simulink model "lss"  (R2022b)
settings: Solver=FixedStepAuto  StartTime=0.0  StopTime=Inf  FixedStep=0.001  RelTol=1e-3  EnableMultiTasking=on
InitFcn:
  | clear mex
model workspace (MAT data in the model file):
  worldsim_instance : object (value not decoded)
values from neighbouring files (symbols this model uses):
  ADAS_Control_Mode = 1    [LSS_parameters.m]    (also in lss_ini_param.sldd = 1.0)
  butter_a = 1.0 -1.9911142922016536 0.99115359586893548    [lss_ini_param.sldd]
  butter_a_lka_out = 1.0 -1.5610180758007179 0.641351538057563    [lss_ini_param.sldd]
  butter_b = 9.825916820482009E-6 1.9651833640964018E-5 9.825916820482009E-6    [lss_ini_param.sldd]
  butter_b_lka_out = 0.020083365564211246 0.040166731128422492 0.020083365564211246    [lss_ini_param.sldd]
  index_variant_approaching_speed = 3.0    [lss_ini_param.sldd]
  initCond = vi_worldsim_load_scenario(worldsim_process,scenario_path,'lss_online')    [launcher.m]
  LDW_Activity_Flag = 1    [LSS_parameters.m]    (also in lss_ini_param.sldd = 1.0)
  LDW_Freq_Hz = Sensor_Freq_worldsim    [LSS_parameters.m]    (also in lss_ini_param.sldd = 50.0)
  LDW_LaneGap_dydt_Warning = 50    [LSS_parameters.m]    (also in lss_ini_param.sldd = 50.0)
  LDW_LaneGap_Warning = [0.5 0.25]    [LSS_parameters.m]    (also in lss_ini_param.sldd = 0.5 0.25)
  LDW_Min_Speed = 60    [LSS_parameters.m]    (also in lss_ini_param.sldd = 60.0)
  LDW_Steer_Vibration_Amplitude = 5    [LSS_parameters.m]    (also in lss_ini_param.sldd = 5.0)
  LDW_Steer_Vibration_Freq = 25    [LSS_parameters.m]    (also in lss_ini_param.sldd = 25.0)
  LKA_Activity_Flag = 1    [LSS_parameters.m]    (also in lss_ini_param.sldd = 1.0)
  LKA_D = [0.2 0.3]    [LSS_parameters.m]    (also in lss_ini_param.sldd = 0.2 0.3)
  LKA_Dyn_Rate_Limiter_Gain = 0.1    [LSS_parameters.m]    (also in lss_ini_param.sldd)
  LKA_Dyn_Rate_Limiter_Power = 10    [LSS_parameters.m]    (also in lss_ini_param.sldd = 10.0)
  LKA_Error_dydt_Off = 1    [LSS_parameters.m]    (also in lss_ini_param.sldd = 1.0)
  LKA_Error_Max = 3    [LSS_parameters.m]    (also in lss_ini_param.sldd = 3.0)
  LKA_Error_Off = 0.5    [LSS_parameters.m]    (also in lss_ini_param.sldd)
  LKA_Freq_Hz = Sensor_Freq_worldsim    [LSS_parameters.m]    (also in lss_ini_param.sldd = 50.0)
  LKA_I = [0.025 0.05]    [LSS_parameters.m]    (also in lss_ini_param.sldd = 0.025 0.05)
  LKA_Lane_Gap_Activate = [0.25 0.125]    [LSS_parameters.m]    (also in lss_ini_param.sldd = -0.05 0.125)
  LKA_Lane_Gap_dydt_Activate = 50    [LSS_parameters.m]    (also in lss_ini_param.sldd = 50.0)
  LKA_Min_Speed = 60    [LSS_parameters.m]    (also in lss_ini_param.mat = 50; lss_ini_param.sldd = 50.0)
  LKA_On_Display_Freq = 5    [LSS_parameters.m]    (also in lss_ini_param.sldd = 5.0)
  LKA_P = [0.1 0.2]    [LSS_parameters.m]    (also in lss_ini_param.sldd = 0.1 0.2)
  LKA_Steer_Rate_Max_radps = 1    [LSS_parameters.m]    (also in lss_ini_param.sldd = 1.0)
  radar_source = 2    [LSS_parameters.m]    (also in lss_ini_param.sldd = 2.0)
  Sensor_Freq_worldsim = 50    [launcher.m]    (also in lss_ini_param.sldd = 50.0)
  simulation_crt = '../VI-CarRealTime_model/SedanCar_WorldSim_Offline_send_svm.xml'    [launcher.m]
  stop_number_collisions = 5    [launcher.m]
  stop_speed = 0.001    [launcher.m]
  stop_time = 20    [launcher.m]
  target_speed = 72    [LSS_parameters.m]    (also in launcher.m = initCond.initialVelocity * 3.6)
  variant_approaching_speed = v_lat    [launcher.m]    (also in lss_ini_param.sldd = 0.2 0.3 0.4 0.5 0.6)
  vehicle_width = 1.86    [LSS_parameters.m]    (also in lss_ini_param.sldd = 2.05)
undefined symbols (not defined in the file or in its folder): Driver_Demands, light_brake_center, light_brake_left, light_brake_right, steer_assist, vicrt_initcallback, vicrt_initmexcallback, vicrt_simulationmanager
libraries: simulink x39, simwbSfunlib x15, viworldsim_lib x5
(part 4 of 6)

== system lss/VI-CarRealTime/Output_Bus/adapter ==
  inputBus : Inport
  adaBCre : BusCreator  Inputs=1353
  adaDemux : Demux  Outputs=1353
  adaSel : BusToVector
  outputBus : Outport
  wires:
  inputBus/1 -> adaSel/1
  adaSel/1 -> adaDemux/1
  adaDemux/1 -> adaBCre/1  "aero_forces:aero_balance"
  adaDemux/2 -> adaBCre/2  "aero_forces:center_downforce"
  adaDemux/3 -> adaBCre/3  "aero_forces:center_sideforce"
  adaDemux/4 -> adaBCre/4  "aero_forces:drag_arm"
  adaDemux/5 -> adaBCre/5  "aero_forces:drag_force"
  adaDemux/6 -> adaBCre/6  "aero_forces:drag_force_front"
  adaDemux/7 -> adaBCre/7  "aero_forces:drag_force_rear"
  adaDemux/8 -> adaBCre/8  "aero_forces:drag_torque"
  adaDemux/9 -> adaBCre/9  "aero_forces:front_downforce"
  adaDemux/10 -> adaBCre/10  "aero_forces:front_sideforce"
  adaDemux/11 -> adaBCre/11  "aero_forces:height_auxiliary"
  adaDemux/12 -> adaBCre/12  "aero_forces:height_front"
  adaDemux/13 -> adaBCre/13  "aero_forces:height_rear"
  adaDemux/14 -> adaBCre/14  "aero_forces:lateral_velocity"
  adaDemux/15 -> adaBCre/15  "aero_forces:longitudinal_velocity"
  adaDemux/16 -> adaBCre/16  "aero_forces:pitch"
  adaDemux/17 -> adaBCre/17  "aero_forces:rear_downforce"
  adaDemux/18 -> adaBCre/18  "aero_forces:rear_sideforce"
  adaDemux/19 -> adaBCre/19  "aero_forces:roll"
  adaDemux/20 -> adaBCre/20  "aero_forces:roll_torque"
  adaDemux/21 -> adaBCre/21  "aero_forces:side_slip"
  adaDemux/22 -> adaBCre/22  "aero_forces:steer"
  adaDemux/23 -> adaBCre/23  "aero_forces:vertical_velocity"
  adaDemux/24 -> adaBCre/24  "aero_forces:yaw_torque"
  adaDemux/25 -> adaBCre/25  "Brake:ABS_Activity:L1"
  adaDemux/26 -> adaBCre/26  "Brake:ABS_Activity:L2"
  adaDemux/27 -> adaBCre/27  "Brake:ABS_Activity:R1"
  adaDemux/28 -> adaBCre/28  "Brake:ABS_Activity:R2"
  adaDemux/29 -> adaBCre/29  "Brake:Brake_Moment:L1"
  adaDemux/30 -> adaBCre/30  "Brake:Brake_Moment:L2"
  adaDemux/31 -> adaBCre/31  "Brake:Brake_Moment:R1"
  adaDemux/32 -> adaBCre/32  "Brake:Brake_Moment:R2"
  adaDemux/33 -> adaBCre/33  "Brake:Chamber_Pressure:L1"
  adaDemux/34 -> adaBCre/34  "Brake:Chamber_Pressure:L2"
  adaDemux/35 -> adaBCre/35  "Brake:Chamber_Pressure:R1"
  adaDemux/36 -> adaBCre/36  "Brake:Chamber_Pressure:R2"
  adaDemux/37 -> adaBCre/37  "Brake:Locked_Damper_Moment:L1"
  adaDemux/38 -> adaBCre/38  "Brake:Locked_Damper_Moment:L2"
  adaDemux/39 -> adaBCre/39  "Brake:Locked_Damper_Moment:R1"
  adaDemux/40 -> adaBCre/40  "Brake:Locked_Damper_Moment:R2"
  adaDemux/41 -> adaBCre/41  "Brake:Locked_Moment:L1"
  adaDemux/42 -> adaBCre/42  "Brake:Locked_Moment:L2"
  adaDemux/43 -> adaBCre/43  "Brake:Locked_Moment:R1"
  adaDemux/44 -> adaBCre/44  "Brake:Locked_Moment:R2"
  adaDemux/45 -> adaBCre/45  "Brake:Locked_Spring_Moment:L1"
  adaDemux/46 -> adaBCre/46  "Brake:Locked_Spring_Moment:L2"
  adaDemux/47 -> adaBCre/47  "Brake:Locked_Spring_Moment:R1"
  adaDemux/48 -> adaBCre/48  "Brake:Locked_Spring_Moment:R2"
  adaDemux/49 -> adaBCre/49  "Brake:Locked_Switch:L1"
  adaDemux/50 -> adaBCre/50  "Brake:Locked_Switch:L2"
  adaDemux/51 -> adaBCre/51  "Brake:Locked_Switch:R1"
  adaDemux/52 -> adaBCre/52  "Brake:Locked_Switch:R2"
  adaDemux/53 -> adaBCre/53  "Brake:Lockup_Rotation:L1"
  adaDemux/54 -> adaBCre/54  "Brake:Lockup_Rotation:L2"
  adaDemux/55 -> adaBCre/55  "Brake:Lockup_Rotation:R1"
  adaDemux/56 -> adaBCre/56  "Brake:Lockup_Rotation:R2"
  adaDemux/57 -> adaBCre/57  "bul_jounce_stop_data:force_front"
  adaDemux/58 -> adaBCre/58  "bul_jounce_stop_data:force_rear"
  adaDemux/59 -> adaBCre/59  "bul_jounce_stop_data:jounce_front"
  adaDemux/60 -> adaBCre/60  "bul_jounce_stop_data:jounce_rear"
  adaDemux/61 -> adaBCre/61  "bul_jounce_stop_data:velocity_front"
  adaDemux/62 -> adaBCre/62  "bul_jounce_stop_data:velocity_rear"
  adaDemux/63 -> adaBCre/63  "bul_rebound_stop_data:force_front"
  adaDemux/64 -> adaBCre/64  "bul_rebound_stop_data:force_rear"
  adaDemux/65 -> adaBCre/65  "bul_rebound_stop_data:jounce_front"
  adaDemux/66 -> adaBCre/66  "bul_rebound_stop_data:jounce_rear"
  adaDemux/67 -> adaBCre/67  "bul_rebound_stop_data:velocity_front"
  adaDemux/68 -> adaBCre/68  "bul_rebound_stop_data:velocity_rear"
  adaDemux/69 -> adaBCre/69  "bur_jounce_stop_data:force_front"
  adaDemux/70 -> adaBCre/70  "bur_jounce_stop_data:force_rear"
  adaDemux/71 -> adaBCre/71  "bur_jounce_stop_data:jounce_front"
  adaDemux/72 -> adaBCre/72  "bur_jounce_stop_data:jounce_rear"
  adaDemux/73 -> adaBCre/73  "bur_jounce_stop_data:velocity_front"
  adaDemux/74 -> adaBCre/74  "bur_jounce_stop_data:velocity_rear"
  adaDemux/75 -> adaBCre/75  "bur_rebound_stop_data:force_front"
  adaDemux/76 -> adaBCre/76  "bur_rebound_stop_data:force_rear"
  adaDemux/77 -> adaBCre/77  "bur_rebound_stop_data:jounce_front"
  adaDemux/78 -> adaBCre/78  "bur_rebound_stop_data:jounce_rear"
  adaDemux/79 -> adaBCre/79  "bur_rebound_stop_data:velocity_front"
  adaDemux/80 -> adaBCre/80  "bur_rebound_stop_data:velocity_rear"
  adaDemux/81 -> adaBCre/81  "bus_dmp_jounce_stop_data:displacement_front"
  adaDemux/82 -> adaBCre/82  "bus_dmp_jounce_stop_data:displacement_rear"
  adaDemux/83 -> adaBCre/83  "bus_dmp_jounce_stop_data:force_front"
  adaDemux/84 -> adaBCre/84  "bus_dmp_jounce_stop_data:force_rear"
  adaDemux/85 -> adaBCre/85  "bus_dmp_jounce_stop_data:velocity_front"
  adaDemux/86 -> adaBCre/86  "bus_dmp_jounce_stop_data:velocity_rear"
  adaDemux/87 -> adaBCre/87  "bus_ins_jounce_stop_data:displacement_front"
  adaDemux/88 -> adaBCre/88  "bus_ins_jounce_stop_data:displacement_rear"
  adaDemux/89 -> adaBCre/89  "bus_ins_jounce_stop_data:force_front"
  adaDemux/90 -> adaBCre/90  "bus_ins_jounce_stop_data:force_rear"
  adaDemux/91 -> adaBCre/91  "bus_ins_jounce_stop_data:velocity_front"
  adaDemux/92 -> adaBCre/92  "bus_ins_jounce_stop_data:velocity_rear"
  adaDemux/93 -> adaBCre/93  "bus_roll_dmp_jounce_stop_data:displacement_front"
  adaDemux/94 -> adaBCre/94  "bus_roll_dmp_jounce_stop_data:displacement_rear"
  adaDemux/95 -> adaBCre/95  "bus_roll_dmp_jounce_stop_data:force_front"
  adaDemux/96 -> adaBCre/96  "bus_roll_dmp_jounce_stop_data:force_rear"
  adaDemux/97 -> adaBCre/97  "bus_roll_dmp_jounce_stop_data:velocity_front"
  adaDemux/98 -> adaBCre/98  "bus_roll_dmp_jounce_stop_data:velocity_rear"
  adaDemux/99 -> adaBCre/99  "bus_spr_jounce_stop_data:displacement_front"
  adaDemux/100 -> adaBCre/100  "bus_spr_jounce_stop_data:displacement_rear"
  adaDemux/101 -> adaBCre/101  "bus_spr_jounce_stop_data:force_front"
  adaDemux/102 -> adaBCre/102  "bus_spr_jounce_stop_data:force_rear"
  adaDemux/103 -> adaBCre/103  "bus_spr_jounce_stop_data:velocity_front"
  adaDemux/104 -> adaBCre/104  "bus_spr_jounce_stop_data:velocity_rear"
  adaDemux/105 -> adaBCre/105  "chassis_accelerations:lateral"
  adaDemux/106 -> adaBCre/106  "chassis_accelerations:longitudinal"
  adaDemux/107 -> adaBCre/107  "chassis_accelerations:pitch"
  adaDemux/108 -> adaBCre/108  "chassis_accelerations:roll"
  adaDemux/109 -> adaBCre/109  "chassis_accelerations:vertical"
  adaDemux/110 -> adaBCre/110  "chassis_accelerations:yaw"
  adaDemux/111 -> adaBCre/111  "chassis_displacements:lateral"
  adaDemux/112 -> adaBCre/112  "chassis_displacements:longitudinal"
  adaDemux/113 -> adaBCre/113  "chassis_displacements:pitch"
  adaDemux/114 -> adaBCre/114  "chassis_displacements:pitch_wrt_road"
  adaDemux/115 -> adaBCre/115  "chassis_displacements:roll"
  adaDemux/116 -> adaBCre/116  "chassis_displacements:roll_wrt_road"
  adaDemux/117 -> adaBCre/117  "chassis_displacements:vertical"
  adaDemux/118 -> adaBCre/118  "chassis_displacements:vertical_wrt_road"
  adaDemux/119 -> adaBCre/119  "chassis_displacements:yaw"
  adaDemux/120 -> adaBCre/120  "chassis_velocities:lateral"
  adaDemux/121 -> adaBCre/121  "chassis_velocities:longitudinal"
  adaDemux/122 -> adaBCre/122  "chassis_velocities:pitch"
  adaDemux/123 -> adaBCre/123  "chassis_velocities:roll"
  adaDemux/124 -> adaBCre/124  "chassis_velocities:vertical"
  adaDemux/125 -> adaBCre/125  "chassis_velocities:yaw"
  adaDemux/126 -> adaBCre/126  "clutch:clutch_rpm"
  adaDemux/127 -> adaBCre/127  "clutch:effective_clutch"
  adaDemux/128 -> adaBCre/128  "clutch:gearbox_inputshaft_alpha"
  adaDemux/129 -> adaBCre/129  "clutch:gearbox_inputshaft_angle"
  adaDemux/130 -> adaBCre/130  "clutch:gearbox_inputshaft_omega"
  adaDemux/131 -> adaBCre/131  "clutch:inputplate_torque"
  adaDemux/132 -> adaBCre/132  "clutch:slip_angle"
  adaDemux/133 -> adaBCre/133  "clutch:torque"
  adaDemux/134 -> adaBCre/134  "condition_sensors:side_slip_angle"
  adaDemux/135 -> adaBCre/135  "cross_weight:crossL1R2_ratio"
  adaDemux/136 -> adaBCre/136  "cross_weight:crossR1L2_ratio"
  adaDemux/137 -> adaBCre/137  "cross_weight:nose_ratio"
  adaDemux/138 -> adaBCre/138  "cross_weight:side_right_ratio"
  adaDemux/139 -> adaBCre/139  "dal_ride_damper_data:force_front"
  adaDemux/140 -> adaBCre/140  "dal_ride_damper_data:force_rear"
  adaDemux/141 -> adaBCre/141  "dal_ride_damper_data:velocity_front"
  adaDemux/142 -> adaBCre/142  "dal_ride_damper_data:velocity_rear"
  adaDemux/143 -> adaBCre/143  "Damper:Force_At_Damper:L1"
  adaDemux/144 -> adaBCre/144  "Damper:Force_At_Damper:L2"
  adaDemux/145 -> adaBCre/145  "Damper:Force_At_Damper:R1"
  adaDemux/146 -> adaBCre/146  "Damper:Force_At_Damper:R2"
  adaDemux/147 -> adaBCre/147  "Damper:Force_At_Wheel:L1"
  adaDemux/148 -> adaBCre/148  "Damper:Force_At_Wheel:L2"
  adaDemux/149 -> adaBCre/149  "Damper:Force_At_Wheel:R1"
  adaDemux/150 -> adaBCre/150  "Damper:Force_At_Wheel:R2"
  adaDemux/151 -> adaBCre/151  "Damper:Jounce:L1"
  adaDemux/152 -> adaBCre/152  "Damper:Jounce:L2"
  adaDemux/153 -> adaBCre/153  "Damper:Jounce:R1"
  adaDemux/154 -> adaBCre/154  "Damper:Jounce:R2"
  adaDemux/155 -> adaBCre/155  "Damper:Jounce_Acceleration:L1"
  adaDemux/156 -> adaBCre/156  "Damper:Jounce_Acceleration:L2"
  adaDemux/157 -> adaBCre/157  "Damper:Jounce_Acceleration:R1"
  adaDemux/158 -> adaBCre/158  "Damper:Jounce_Acceleration:R2"
  adaDemux/159 -> adaBCre/159  "Damper:Jounce_Rate:L1"
  adaDemux/160 -> adaBCre/160  "Damper:Jounce_Rate:L2"
  adaDemux/161 -> adaBCre/161  "Damper:Jounce_Rate:R1"
  adaDemux/162 -> adaBCre/162  "Damper:Jounce_Rate:R2"
  adaDemux/163 -> adaBCre/163  "dar_ride_damper_data:force_front"
  adaDemux/164 -> adaBCre/164  "dar_ride_damper_data:force_rear"
  adaDemux/165 -> adaBCre/165  "dar_ride_damper_data:velocity_front"
  adaDemux/166 -> adaBCre/166  "dar_ride_damper_data:velocity_rear"
  adaDemux/167 -> adaBCre/167  "das_ride_damper_data:displacement_front"
  adaDemux/168 -> adaBCre/168  "das_ride_damper_data:displacement_rear"
  adaDemux/169 -> adaBCre/169  "das_ride_damper_data:force_front"
  adaDemux/170 -> adaBCre/170  "das_ride_damper_data:force_rear"
  adaDemux/171 -> adaBCre/171  "das_ride_damper_data:velocity_front"
  adaDemux/172 -> adaBCre/172  "das_ride_damper_data:velocity_rear"
  adaDemux/173 -> adaBCre/173  "das_roll_damper_data:displacement_front"
  adaDemux/174 -> adaBCre/174  "das_roll_damper_data:displacement_rear"
  adaDemux/175 -> adaBCre/175  "das_roll_damper_data:force_at_wheel_front"
  adaDemux/176 -> adaBCre/176  "das_roll_damper_data:force_at_wheel_rear"
  adaDemux/177 -> adaBCre/177  "das_roll_damper_data:force_front"
  adaDemux/178 -> adaBCre/178  "das_roll_damper_data:force_rear"
  adaDemux/179 -> adaBCre/179  "das_roll_damper_data:velocity_front"
  adaDemux/180 -> adaBCre/180  "das_roll_damper_data:velocity_rear"
  adaDemux/181 -> adaBCre/181  "das_third_damper_data:displacement_front"
  adaDemux/182 -> adaBCre/182  "das_third_damper_data:displacement_rear"
  adaDemux/183 -> adaBCre/183  "das_third_damper_data:force_front"
  adaDemux/184 -> adaBCre/184  "das_third_damper_data:force_rear"
  adaDemux/185 -> adaBCre/185  "das_third_damper_data:velocity_front"
  adaDemux/186 -> adaBCre/186  "das_third_damper_data:velocity_rear"
  adaDemux/187 -> adaBCre/187  "differential_central:diff_front_inputshaft_alpha"
  adaDemux/188 -> adaBCre/188  "differential_central:diff_front_inputshaft_angle"
  adaDemux/189 -> adaBCre/189  "differential_central:diff_front_inputshaft_omega"
  adaDemux/190 -> adaBCre/190  "differential_central:diff_rear_inputshaft_alpha"
  adaDemux/191 -> adaBCre/191  "differential_central:diff_rear_inputshaft_angle"
  adaDemux/192 -> adaBCre/192  "differential_central:diff_rear_inputshaft_omega"
  adaDemux/193 -> adaBCre/193  "differential_central:gearbox_outputshaft_torque"
  adaDemux/194 -> adaBCre/194  "differential_front:diff_central_front_outputshaft_torque"
  adaDemux/195 -> adaBCre/195  "differential_front:wheel_front_left_alpha"
  adaDemux/196 -> adaBCre/196  "differential_front:wheel_front_left_angle"
  adaDemux/197 -> adaBCre/197  "differential_front:wheel_front_left_omega"
  adaDemux/198 -> adaBCre/198  "differential_front:wheel_front_right_alpha"
  adaDemux/199 -> adaBCre/199  "differential_front:wheel_front_right_angle"
  adaDemux/200 -> adaBCre/200  "differential_front:wheel_front_right_omega"
  adaDemux/201 -> adaBCre/201  "differential_rear:diff_central_rear_outputshaft_torque"
  adaDemux/202 -> adaBCre/202  "differential_rear:wheel_rear_left_alpha"
  adaDemux/203 -> adaBCre/203  "differential_rear:wheel_rear_left_angle"
  adaDemux/204 -> adaBCre/204  "differential_rear:wheel_rear_left_omega"
  adaDemux/205 -> adaBCre/205  "differential_rear:wheel_rear_right_alpha"
  adaDemux/206 -> adaBCre/206  "differential_rear:wheel_rear_right_angle"
  adaDemux/207 -> adaBCre/207  "differential_rear:wheel_rear_right_omega"
  adaDemux/208 -> adaBCre/208  "differential_speeds:halfshaft_omega_central_front"
  adaDemux/209 -> adaBCre/209  "differential_speeds:halfshaft_omega_central_rear"
  adaDemux/210 -> adaBCre/210  "differential_speeds:halfshaft_omega_delta_central"
  adaDemux/211 -> adaBCre/211  "differential_speeds:halfshaft_omega_delta_front"
  adaDemux/212 -> adaBCre/212  "differential_speeds:halfshaft_omega_delta_rear"
  adaDemux/213 -> adaBCre/213  "differential_speeds:halfshaft_omega_left_front"
  adaDemux/214 -> adaBCre/214  "differential_speeds:halfshaft_omega_left_rear"
  adaDemux/215 -> adaBCre/215  "differential_speeds:halfshaft_omega_right_front"
  adaDemux/216 -> adaBCre/216  "differential_speeds:halfshaft_omega_right_rear"
  adaDemux/217 -> adaBCre/217  "differential_torques:differential_torque_central"
  adaDemux/218 -> adaBCre/218  "differential_torques:differential_torque_front"
  adaDemux/219 -> adaBCre/219  "differential_torques:differential_torque_rear"
  adaDemux/220 -> adaBCre/220  "differential_torques:output_torque_central_front"
  adaDemux/221 -> adaBCre/221  "differential_torques:output_torque_central_rear"
  adaDemux/222 -> adaBCre/222  "differential_torques:output_torque_left_front"
  adaDemux/223 -> adaBCre/223  "differential_torques:output_torque_left_rear"
  adaDemux/224 -> adaBCre/224  "differential_torques:output_torque_right_front"
  adaDemux/225 -> adaBCre/225  "differential_torques:output_torque_right_rear"
  adaDemux/226 -> adaBCre/226  "driver_demands:brake"
  adaDemux/227 -> adaBCre/227  "driver_demands:brake_pressure"
  adaDemux/228 -> adaBCre/228  "driver_demands:clutch"
  adaDemux/229 -> adaBCre/229  "driver_demands:gear"
  adaDemux/230 -> adaBCre/230  "driver_demands:steering"
  adaDemux/231 -> adaBCre/231  "driver_demands:steering_velocity"
  adaDemux/232 -> adaBCre/232  "driver_demands:throttle"
  adaDemux/233 -> adaBCre/233  "driver_demands:steering_acceleration"
  adaDemux/234 -> adaBCre/234  "driver_demands:driver_steering_angle"
  adaDemux/235 -> adaBCre/235  "driving_machine_monitor:driver_brake"
  adaDemux/236 -> adaBCre/236  "driving_machine_monitor:driver_clutch"
  adaDemux/237 -> adaBCre/237  "driving_machine_monitor:driver_gear"
  adaDemux/238 -> adaBCre/238  "driving_machine_monitor:driver_steering"
  adaDemux/239 -> adaBCre/239  "driving_machine_monitor:driver_throttle"
  adaDemux/240 -> adaBCre/240  "driving_machine_monitor:maneuver_ID"
  adaDemux/241 -> adaBCre/241  "driving_machine_monitor:path_curvature"
  adaDemux/242 -> adaBCre/242  "driving_machine_monitor:path_distance"
  adaDemux/243 -> adaBCre/243  "driving_machine_monitor:path_s"
  adaDemux/244 -> adaBCre/244  "driving_machine_monitor:path_x"
  adaDemux/245 -> adaBCre/245  "driving_machine_monitor:path_y"
  adaDemux/246 -> adaBCre/246  "driving_machine_monitor:path_z"
  adaDemux/247 -> adaBCre/247  "driving_machine_monitor:target_ax"
  adaDemux/248 -> adaBCre/248  "driving_machine_monitor:target_engine_torque"
  adaDemux/249 -> adaBCre/249  "driving_machine_monitor:target_vx"
  adaDemux/250 -> adaBCre/250  "engine:clutch_inputplate_alpha"
  adaDemux/251 -> adaBCre/251  "engine:clutch_inputplate_angle"
  adaDemux/252 -> adaBCre/252  "engine:clutch_inputplate_omega"
  adaDemux/253 -> adaBCre/253  "engine:effective_throttle"
  adaDemux/254 -> adaBCre/254  "engine:engine_rpm"
  adaDemux/255 -> adaBCre/255  "engine:Max_Engine_torque"
  adaDemux/256 -> adaBCre/256  "engine:Min_engine_torque"
  adaDemux/257 -> adaBCre/257  "engine:Power_HP"
  adaDemux/258 -> adaBCre/258  "engine:Power_KW"
  adaDemux/259 -> adaBCre/259  "engine:TCS_activity"
  adaDemux/260 -> adaBCre/260  "engine:torque"
  adaDemux/261 -> adaBCre/261  "fuel_consumption:BSFC"
  adaDemux/262 -> adaBCre/262  "fuel_consumption:instantaneous"
  adaDemux/263 -> adaBCre/263  "fuel_consumption:instantaneous_Liter_100km"
  adaDemux/264 -> adaBCre/264  "fuel_consumption:overall"
  adaDemux/265 -> adaBCre/265  "fuel_consumption:fuel_mass"
  adaDemux/266 -> adaBCre/266  "ges_chassis_XFORM:Phi"
  adaDemux/267 -> adaBCre/267  "ges_chassis_XFORM:Psi"
  adaDemux/268 -> adaBCre/268  "ges_chassis_XFORM:Theta"
  adaDemux/269 -> adaBCre/269  "ges_chassis_XFORM:X"
  adaDemux/270 -> adaBCre/270  "ges_chassis_XFORM:Y"
  adaDemux/271 -> adaBCre/271  "ges_chassis_XFORM:Z"
  adaDemux/272 -> adaBCre/272  "Gyro:Driver_X"
  adaDemux/273 -> adaBCre/273  "Gyro:Driver_Z"
  adaDemux/274 -> adaBCre/274  "Gyro:gyro_ACCX"
  adaDemux/275 -> adaBCre/275  "Gyro:gyro_ACCY"
  adaDemux/276 -> adaBCre/276  "Gyro:gyro_VX"
  adaDemux/277 -> adaBCre/277  "Gyro:gyro_X"
  adaDemux/278 -> adaBCre/278  "Gyro:gyro_Y"
  adaDemux/279 -> adaBCre/279  "Gyro:sensor_1_Z"
  adaDemux/280 -> adaBCre/280  "Gyro:sensor_2_Z"
  adaDemux/281 -> adaBCre/281  "Gyro:sensor_3_Z"
  adaDemux/282 -> adaBCre/282  "Hook_rear:Global_force_X"
  adaDemux/283 -> adaBCre/283  "Hook_rear:Global_force_Y"
  adaDemux/284 -> adaBCre/284  "Hook_rear:Global_force_Z"
  adaDemux/285 -> adaBCre/285  "Hook_rear:Global_Moment_X"
  adaDemux/286 -> adaBCre/286  "Hook_rear:Global_Moment_Y"
  adaDemux/287 -> adaBCre/287  "Hook_rear:Global_Moment_Z"
  adaDemux/288 -> adaBCre/288  "Hook_rear:Hook_Phi"
  adaDemux/289 -> adaBCre/289  "Hook_rear:Hook_Psi"
  adaDemux/290 -> adaBCre/290  "Hook_rear:Hook_Theta"
  adaDemux/291 -> adaBCre/291  "Hook_rear:Hook_X"
  adaDemux/292 -> adaBCre/292  "Hook_rear:Hook_Y"
  adaDemux/293 -> adaBCre/293  "Hook_rear:Hook_Z"
  adaDemux/294 -> adaBCre/294  "Hook_rear:Local_force_X"
  adaDemux/295 -> adaBCre/295  "Hook_rear:Local_force_Y"
  adaDemux/296 -> adaBCre/296  "Hook_rear:Local_force_Z"
  adaDemux/297 -> adaBCre/297  "Hook_rear:Local_Moment_X"
  adaDemux/298 -> adaBCre/298  "Hook_rear:Local_Moment_Y"
  adaDemux/299 -> adaBCre/299  "Hook_rear:Local_Moment_Z"
  adaDemux/300 -> adaBCre/300  "Inerter:Force_At_Inerter:L1"
  adaDemux/301 -> adaBCre/301  "Inerter:Force_At_Inerter:L2"
  adaDemux/302 -> adaBCre/302  "Inerter:Force_At_Inerter:R1"
  adaDemux/303 -> adaBCre/303  "Inerter:Force_At_Inerter:R2"
  adaDemux/304 -> adaBCre/304  "Inerter:Force_At_Wheel:L1"
  adaDemux/305 -> adaBCre/305  "Inerter:Force_At_Wheel:L2"
  adaDemux/306 -> adaBCre/306  "Inerter:Force_At_Wheel:R1"
  adaDemux/307 -> adaBCre/307  "Inerter:Force_At_Wheel:R2"
  adaDemux/308 -> adaBCre/308  "Inerter:Jounce:L1"
  adaDemux/309 -> adaBCre/309  "Inerter:Jounce:L2"
  adaDemux/310 -> adaBCre/310  "Inerter:Jounce:R1"
  adaDemux/311 -> adaBCre/311  "Inerter:Jounce:R2"
  adaDemux/312 -> adaBCre/312  "Inerter:Jounce_Acceleration:L1"
  adaDemux/313 -> adaBCre/313  "Inerter:Jounce_Acceleration:L2"
  adaDemux/314 -> adaBCre/314  "Inerter:Jounce_Acceleration:R1"
  adaDemux/315 -> adaBCre/315  "Inerter:Jounce_Acceleration:R2"
  adaDemux/316 -> adaBCre/316  "Inerter:Jounce_Rate:L1"
  adaDemux/317 -> adaBCre/317  "Inerter:Jounce_Rate:L2"
  adaDemux/318 -> adaBCre/318  "Inerter:Jounce_Rate:R1"
  adaDemux/319 -> adaBCre/319  "Inerter:Jounce_Rate:R2"
  adaDemux/320 -> adaBCre/320  "inl_ride_inerter_data:acceleration_front"
  adaDemux/321 -> adaBCre/321  "inl_ride_inerter_data:acceleration_rear"
  adaDemux/322 -> adaBCre/322  "inl_ride_inerter_data:displacement_front"
  adaDemux/323 -> adaBCre/323  "inl_ride_inerter_data:displacement_rear"
  adaDemux/324 -> adaBCre/324  "inl_ride_inerter_data:force_front"
  adaDemux/325 -> adaBCre/325  "inl_ride_inerter_data:force_rear"
  adaDemux/326 -> adaBCre/326  "inr_ride_inerter_data:acceleration_front"
  adaDemux/327 -> adaBCre/327  "inr_ride_inerter_data:acceleration_rear"
  adaDemux/328 -> adaBCre/328  "inr_ride_inerter_data:displacement_front"
  adaDemux/329 -> adaBCre/329  "inr_ride_inerter_data:displacement_rear"
  adaDemux/330 -> adaBCre/330  "inr_ride_inerter_data:force_front"
  adaDemux/331 -> adaBCre/331  "inr_ride_inerter_data:force_rear"
  adaDemux/332 -> adaBCre/332  "ins_inerter_data:acceleration_front"
  adaDemux/333 -> adaBCre/333  "ins_inerter_data:acceleration_rear"
  adaDemux/334 -> adaBCre/334  "ins_inerter_data:displacement_front"
  adaDemux/335 -> adaBCre/335  "ins_inerter_data:displacement_rear"
  adaDemux/336 -> adaBCre/336  "ins_inerter_data:force_at_wheel_front"
  adaDemux/337 -> adaBCre/337  "ins_inerter_data:force_at_wheel_rear"
  adaDemux/338 -> adaBCre/338  "ins_inerter_data:force_front"
  adaDemux/339 -> adaBCre/339  "ins_inerter_data:force_rear"
  adaDemux/340 -> adaBCre/340  "ins_inerter_data:velocity_front"
  adaDemux/341 -> adaBCre/341  "ins_inerter_data:velocity_rear"
  adaDemux/342 -> adaBCre/342  "jfs_torsional_stiffness_data:AX_1"
  adaDemux/343 -> adaBCre/343  "jfs_torsional_stiffness_data:AY_1"
  adaDemux/344 -> adaBCre/344  "jfs_torsional_stiffness_data:AZ_1"
  adaDemux/345 -> adaBCre/345  "jfs_torsional_stiffness_data:FX_1"
  adaDemux/346 -> adaBCre/346  "jfs_torsional_stiffness_data:FY_1"
  adaDemux/347 -> adaBCre/347  "jfs_torsional_stiffness_data:FZ_1"
  adaDemux/348 -> adaBCre/348  "jfs_torsional_stiffness_data:TX_1"
  adaDemux/349 -> adaBCre/349  "jfs_torsional_stiffness_data:TY_1"
  adaDemux/350 -> adaBCre/350  "jfs_torsional_stiffness_data:TZ_1"
  adaDemux/351 -> adaBCre/351  "jfs_torsional_stiffness_data:X_1"
  adaDemux/352 -> adaBCre/352  "jfs_torsional_stiffness_data:Y_1"
  adaDemux/353 -> adaBCre/353  "jfs_torsional_stiffness_data:Z_1"
  adaDemux/354 -> adaBCre/354  "Jounce_Bumper:Force_At_Bumper:L1"
  adaDemux/355 -> adaBCre/355  "Jounce_Bumper:Force_At_Bumper:L2"
  adaDemux/356 -> adaBCre/356  "Jounce_Bumper:Force_At_Bumper:R1"
  adaDemux/357 -> adaBCre/357  "Jounce_Bumper:Force_At_Bumper:R2"
  adaDemux/358 -> adaBCre/358  "Jounce_Bumper:Force_At_Wheel:L1"
  adaDemux/359 -> adaBCre/359  "Jounce_Bumper:Force_At_Wheel:L2"
  adaDemux/360 -> adaBCre/360  "Jounce_Bumper:Force_At_Wheel:R1"
  adaDemux/361 -> adaBCre/361  "Jounce_Bumper:Force_At_Wheel:R2"
  adaDemux/362 -> adaBCre/362  "Jounce_Bumper:Jounce:L1"
  adaDemux/363 -> adaBCre/363  "Jounce_Bumper:Jounce:L2"
  adaDemux/364 -> adaBCre/364  "Jounce_Bumper:Jounce:R1"
  adaDemux/365 -> adaBCre/365  "Jounce_Bumper:Jounce:R2"
  adaDemux/366 -> adaBCre/366  "Jounce_Bumper:Jounce_Rate:L1"
  adaDemux/367 -> adaBCre/367  "Jounce_Bumper:Jounce_Rate:L2"
  adaDemux/368 -> adaBCre/368  "Jounce_Bumper:Jounce_Rate:R1"
  adaDemux/369 -> adaBCre/369  "Jounce_Bumper:Jounce_Rate:R2"
  adaDemux/370 -> adaBCre/370  "nsl_ride_spring_data:displacement_front"
  adaDemux/371 -> adaBCre/371  "nsl_ride_spring_data:displacement_rear"
  adaDemux/372 -> adaBCre/372  "nsl_ride_spring_data:force_front"
  adaDemux/373 -> adaBCre/373  "nsl_ride_spring_data:force_rear"
  adaDemux/374 -> adaBCre/374  "nsl_ride_spring_data:velocity_front"
  adaDemux/375 -> adaBCre/375  "nsl_ride_spring_data:velocity_rear"
  adaDemux/376 -> adaBCre/376  "nsr_ride_spring_data:displacement_front"
  adaDemux/377 -> adaBCre/377  "nsr_ride_spring_data:displacement_rear"
  adaDemux/378 -> adaBCre/378  "nsr_ride_spring_data:force_front"
  adaDemux/379 -> adaBCre/379  "nsr_ride_spring_data:force_rear"
  adaDemux/380 -> adaBCre/380  "nsr_ride_spring_data:velocity_front"
  adaDemux/381 -> adaBCre/381  "nsr_ride_spring_data:velocity_rear"
  adaDemux/382 -> adaBCre/382  "nss_ride_spring_data:displacement_front"
  adaDemux/383 -> adaBCre/383  "nss_ride_spring_data:displacement_rear"
  adaDemux/384 -> adaBCre/384  "nss_ride_spring_data:force_at_wheel_front"
  adaDemux/385 -> adaBCre/385  "nss_ride_spring_data:force_at_wheel_rear"
  adaDemux/386 -> adaBCre/386  "nss_ride_spring_data:force_front"
  adaDemux/387 -> adaBCre/387  "nss_ride_spring_data:force_rear"
  adaDemux/388 -> adaBCre/388  "nss_ride_spring_data:PID_PH_At_Spring_front"
  adaDemux/389 -> adaBCre/389  "nss_ride_spring_data:PID_PH_At_Spring_rear"
  adaDemux/390 -> adaBCre/390  "nss_ride_spring_data:velocity_front"
  adaDemux/391 -> adaBCre/391  "nss_ride_spring_data:velocity_rear"
  adaDemux/392 -> adaBCre/392  "Rebound_Bumper:Force_At_Bumper:L1"
  adaDemux/393 -> adaBCre/393  "Rebound_Bumper:Force_At_Bumper:L2"
  adaDemux/394 -> adaBCre/394  "Rebound_Bumper:Force_At_Bumper:R1"
  adaDemux/395 -> adaBCre/395  "Rebound_Bumper:Force_At_Bumper:R2"
  adaDemux/396 -> adaBCre/396  "Rebound_Bumper:Force_At_Wheel:L1"
  adaDemux/397 -> adaBCre/397  "Rebound_Bumper:Force_At_Wheel:L2"
  adaDemux/398 -> adaBCre/398  "Rebound_Bumper:Force_At_Wheel:R1"
  adaDemux/399 -> adaBCre/399  "Rebound_Bumper:Force_At_Wheel:R2"
  adaDemux/400 -> adaBCre/400  "Rebound_Bumper:Jounce:L1"
  adaDemux/401 -> adaBCre/401  "Rebound_Bumper:Jounce:L2"
  adaDemux/402 -> adaBCre/402  "Rebound_Bumper:Jounce:R1"
  adaDemux/403 -> adaBCre/403  "Rebound_Bumper:Jounce:R2"
  adaDemux/404 -> adaBCre/404  "Rebound_Bumper:Jounce_Rate:L1"
  adaDemux/405 -> adaBCre/405  "Rebound_Bumper:Jounce_Rate:L2"
  adaDemux/406 -> adaBCre/406  "Rebound_Bumper:Jounce_Rate:R1"
  adaDemux/407 -> adaBCre/407  "Rebound_Bumper:Jounce_Rate:R2"
  adaDemux/408 -> adaBCre/408  "res_dmp_rebound_stop_data:displacement_front"
  adaDemux/409 -> adaBCre/409  "res_dmp_rebound_stop_data:displacement_rear"
  adaDemux/410 -> adaBCre/410  "res_dmp_rebound_stop_data:force_front"
  adaDemux/411 -> adaBCre/411  "res_dmp_rebound_stop_data:force_rear"
  adaDemux/412 -> adaBCre/412  "res_dmp_rebound_stop_data:velocity_front"
  adaDemux/413 -> adaBCre/413  "res_dmp_rebound_stop_data:velocity_rear"
  adaDemux/414 -> adaBCre/414  "res_ins_rebound_stop_data:displacement_front"
  adaDemux/415 -> adaBCre/415  "res_ins_rebound_stop_data:displacement_rear"
  adaDemux/416 -> adaBCre/416  "res_ins_rebound_stop_data:force_front"
  adaDemux/417 -> adaBCre/417  "res_ins_rebound_stop_data:force_rear"
  adaDemux/418 -> adaBCre/418  "res_ins_rebound_stop_data:velocity_front"
  adaDemux/419 -> adaBCre/419  "res_ins_rebound_stop_data:velocity_rear"
  adaDemux/420 -> adaBCre/420  "res_roll_dmp_rebound_stop_data:displacement_front"
  adaDemux/421 -> adaBCre/421  "res_roll_dmp_rebound_stop_data:displacement_rear"
  adaDemux/422 -> adaBCre/422  "res_roll_dmp_rebound_stop_data:force_front"
  adaDemux/423 -> adaBCre/423  "res_roll_dmp_rebound_stop_data:force_rear"
  adaDemux/424 -> adaBCre/424  "res_roll_dmp_rebound_stop_data:velocity_front"
  adaDemux/425 -> adaBCre/425  "res_roll_dmp_rebound_stop_data:velocity_rear"
  adaDemux/426 -> adaBCre/426  "res_spr_rebound_stop_data:displacement_front"
  adaDemux/427 -> adaBCre/427  "res_spr_rebound_stop_data:displacement_rear"
  adaDemux/428 -> adaBCre/428  "res_spr_rebound_stop_data:force_front"
  adaDemux/429 -> adaBCre/429  "res_spr_rebound_stop_data:force_rear"
  adaDemux/430 -> adaBCre/430  "res_spr_rebound_stop_data:velocity_front"
  adaDemux/431 -> adaBCre/431  "res_spr_rebound_stop_data:velocity_rear"
  adaDemux/432 -> adaBCre/432  "rhl_front_setup_sensor_data:ride_height"
  adaDemux/433 -> adaBCre/433  "rhl_rear_setup_sensor_data:ride_height"
  adaDemux/434 -> adaBCre/434  "rhr_front_setup_sensor_data:ride_height"
  adaDemux/435 -> adaBCre/435  "rhr_rear_setup_sensor_data:ride_height"
  adaDemux/436 -> adaBCre/436  "rhs_front_setup_sensor_data:ride_height"
  adaDemux/437 -> adaBCre/437  "rhs_rear_setup_sensor_data:ride_height"
  adaDemux/438 -> adaBCre/438  "Road:Contact_Flag:L1"
  adaDemux/439 -> adaBCre/439  "Road:Contact_Flag:L2"
  adaDemux/440 -> adaBCre/440  "Road:Contact_Flag:R1"
  adaDemux/441 -> adaBCre/441  "Road:Contact_Flag:R2"
  adaDemux/442 -> adaBCre/442  "Road:Contact_Patch_Global_X:L1"
  adaDemux/443 -> adaBCre/443  "Road:Contact_Patch_Global_X:L2"
  adaDemux/444 -> adaBCre/444  "Road:Contact_Patch_Global_X:R1"
  adaDemux/445 -> adaBCre/445  "Road:Contact_Patch_Global_X:R2"
  adaDemux/446 -> adaBCre/446  "Road:Contact_Patch_Global_Y:L1"
  adaDemux/447 -> adaBCre/447  "Road:Contact_Patch_Global_Y:L2"
  adaDemux/448 -> adaBCre/448  "Road:Contact_Patch_Global_Y:R1"
  adaDemux/449 -> adaBCre/449  "Road:Contact_Patch_Global_Y:R2"
  adaDemux/450 -> adaBCre/450  "Road:Contact_Patch_Global_Z:L1"
  adaDemux/451 -> adaBCre/451  "Road:Contact_Patch_Global_Z:L2"
  adaDemux/452 -> adaBCre/452  "Road:Contact_Patch_Global_Z:R1"
  adaDemux/453 -> adaBCre/453  "Road:Contact_Patch_Global_Z:R2"
  adaDemux/454 -> adaBCre/454  "Road:Off_Road_Flag:L1"
  adaDemux/455 -> adaBCre/455  "Road:Off_Road_Flag:L2"
  adaDemux/456 -> adaBCre/456  "Road:Off_Road_Flag:R1"
  adaDemux/457 -> adaBCre/457  "Road:Off_Road_Flag:R2"
  adaDemux/458 -> adaBCre/458  "Sensor:AccX_gyro"
  adaDemux/459 -> adaBCre/459  "Sensor:AccY_gyro"
  adaDemux/460 -> adaBCre/460  "Sensor:Ax"
  adaDemux/461 -> adaBCre/461  "Sensor:Ax_Without_Gravity"
  adaDemux/462 -> adaBCre/462  "Sensor:Ay"
  adaDemux/463 -> adaBCre/463  "Sensor:Ay_Without_Gravity"
  adaDemux/464 -> adaBCre/464  "Sensor:Az"
  adaDemux/465 -> adaBCre/465  "Sensor:Az_Without_Gravity"
  adaDemux/466 -> adaBCre/466  "Sensor:Global_X"
  adaDemux/467 -> adaBCre/467  "Sensor:Global_Y"
  adaDemux/468 -> adaBCre/468  "Sensor:Global_Z"
  adaDemux/469 -> adaBCre/469  "Sensor:Vx"
  adaDemux/470 -> adaBCre/470  "Sensor:Vx_gyro"
  adaDemux/471 -> adaBCre/471  "Sensor:Vy"
  adaDemux/472 -> adaBCre/472  "Sensor:Vz"
  adaDemux/473 -> adaBCre/473  "Sensor:YawRate_gyro"
  adaDemux/474 -> adaBCre/474  "Spring:Aggregate_Force_At_Wheel:L1"
  adaDemux/475 -> adaBCre/475  "Spring:Aggregate_Force_At_Wheel:L2"
  adaDemux/476 -> adaBCre/476  "Spring:Aggregate_Force_At_Wheel:R1"
  adaDemux/477 -> adaBCre/477  "Spring:Aggregate_Force_At_Wheel:R2"
  adaDemux/478 -> adaBCre/478  "Spring:Force_At_Spring:L1"
  adaDemux/479 -> adaBCre/479  "Spring:Force_At_Spring:L2"
  adaDemux/480 -> adaBCre/480  "Spring:Force_At_Spring:R1"
  adaDemux/481 -> adaBCre/481  "Spring:Force_At_Spring:R2"
  adaDemux/482 -> adaBCre/482  "Spring:Force_At_Wheel:L1"
  adaDemux/483 -> adaBCre/483  "Spring:Force_At_Wheel:L2"
  adaDemux/484 -> adaBCre/484  "Spring:Force_At_Wheel:R1"
  adaDemux/485 -> adaBCre/485  "Spring:Force_At_Wheel:R2"
  adaDemux/486 -> adaBCre/486  "Spring:Force_Aux_At_Wheel:L1"
  adaDemux/487 -> adaBCre/487  "Spring:Force_Aux_At_Wheel:L2"
  adaDemux/488 -> adaBCre/488  "Spring:Force_Aux_At_Wheel:R1"
  adaDemux/489 -> adaBCre/489  "Spring:Force_Aux_At_Wheel:R2"
  adaDemux/490 -> adaBCre/490  "Spring:Jounce:L1"
  adaDemux/491 -> adaBCre/491  "Spring:Jounce:L2"
  adaDemux/492 -> adaBCre/492  "Spring:Jounce:R1"
  adaDemux/493 -> adaBCre/493  "Spring:Jounce:R2"
  adaDemux/494 -> adaBCre/494  "Spring:Jounce_Acceleration:L1"
  adaDemux/495 -> adaBCre/495  "Spring:Jounce_Acceleration:L2"
  adaDemux/496 -> adaBCre/496  "Spring:Jounce_Acceleration:R1"
  adaDemux/497 -> adaBCre/497  "Spring:Jounce_Acceleration:R2"
  adaDemux/498 -> adaBCre/498  "Spring:Jounce_Rate:L1"
  adaDemux/499 -> adaBCre/499  "Spring:Jounce_Rate:L2"
  adaDemux/500 -> adaBCre/500  "Spring:Jounce_Rate:R1"
  adaDemux/501 -> adaBCre/501  "Spring:Jounce_Rate:R2"
  adaDemux/502 -> adaBCre/502  "Spring:PID_CW_At_Spring:L1"
  adaDemux/503 -> adaBCre/503  "Spring:PID_CW_At_Spring:L2"
  adaDemux/504 -> adaBCre/504  "Spring:PID_CW_At_Spring:R1"
  adaDemux/505 -> adaBCre/505  "Spring:PID_CW_At_Spring:R2"
  adaDemux/506 -> adaBCre/506  "Spring:PID_PH_At_Spring:L1"
  adaDemux/507 -> adaBCre/507  "Spring:PID_PH_At_Spring:L2"
  adaDemux/508 -> adaBCre/508  "Spring:PID_PH_At_Spring:R1"
  adaDemux/509 -> adaBCre/509  "Spring:PID_PH_At_Spring:R2"
  adaDemux/510 -> adaBCre/510  "Spring:PID_RH_At_Spring:L1"
  adaDemux/511 -> adaBCre/511  "Spring:PID_RH_At_Spring:L2"
  adaDemux/512 -> adaBCre/512  "Spring:PID_RH_At_Spring:R1"
  adaDemux/513 -> adaBCre/513  "Spring:PID_RH_At_Spring:R2"
  adaDemux/514 -> adaBCre/514  "Steering_System:DriveSim_Steering_Feedback_Torque"
  adaDemux/515 -> adaBCre/515  "Steering_System:Rack_displacement"
  adaDemux/516 -> adaBCre/516  "Steering_System:Rack_Force"
  adaDemux/517 -> adaBCre/517  "Steering_System:Steering_column_deformation"
  adaDemux/518 -> adaBCre/518  "Steering_System:Steering_Wheel_Torque"
  adaDemux/519 -> adaBCre/519  "Steering_System:TieRod_Force_Left:X"
  adaDemux/520 -> adaBCre/520  "Steering_System:TieRod_Force_Left:Y"
  adaDemux/521 -> adaBCre/521  "Steering_System:TieRod_Force_Left:Z"
  adaDemux/522 -> adaBCre/522  "Steering_System:TieRod_Force_Right:X"
  adaDemux/523 -> adaBCre/523  "Steering_System:TieRod_Force_Right:Y"
  adaDemux/524 -> adaBCre/524  "Steering_System:TieRod_Force_Right:Z"
  adaDemux/525 -> adaBCre/525  "Steering_System:selected_eps_map"
  adaDemux/526 -> adaBCre/526  "Steering_System:eccentricity_torque"
  adaDemux/527 -> adaBCre/527  "Steering_System:pitman_arm_rotation"
  adaDemux/528 -> adaBCre/528  "Steering_System:pitman_arm_saturated_rotation"
  adaDemux/529 -> adaBCre/529  "Steering_System:pitman_arm_velocity"
  adaDemux/530 -> adaBCre/530  "Steering_System:pitman_arm_acceleration"
  adaDemux/531 -> adaBCre/531  "Suspension:Auxiliary_Roll_deformation_at_element:SUSP1"
  adaDemux/532 -> adaBCre/532  "Suspension:Auxiliary_Roll_deformation_at_element:SUSP2"
  adaDemux/533 -> adaBCre/533  "Suspension:Auxiliary_Roll_Force:SUSP_L1"
  adaDemux/534 -> adaBCre/534  "Suspension:Auxiliary_Roll_Force:SUSP_L2"
  adaDemux/535 -> adaBCre/535  "Suspension:Auxiliary_Roll_Force:SUSP_R1"
  adaDemux/536 -> adaBCre/536  "Suspension:Auxiliary_Roll_Force:SUSP_R2"
  adaDemux/537 -> adaBCre/537  "Suspension:Auxiliary_Roll_Force_at_element:SUSP1"
  adaDemux/538 -> adaBCre/538  "Suspension:Auxiliary_Roll_Force_at_element:SUSP2"
  adaDemux/539 -> adaBCre/539  "Suspension:base_acceleration:L1"
  adaDemux/540 -> adaBCre/540  "Suspension:base_acceleration:L2"
  adaDemux/541 -> adaBCre/541  "Suspension:base_acceleration:R1"
  adaDemux/542 -> adaBCre/542  "Suspension:base_acceleration:R2"
  adaDemux/543 -> adaBCre/543  "Suspension:base_deformation:L1"
  adaDemux/544 -> adaBCre/544  "Suspension:base_deformation:L2"
  adaDemux/545 -> adaBCre/545  "Suspension:base_deformation:R1"
  adaDemux/546 -> adaBCre/546  "Suspension:base_deformation:R2"
  adaDemux/547 -> adaBCre/547  "Suspension:base_velocity:L1"
  adaDemux/548 -> adaBCre/548  "Suspension:base_velocity:L2"
  adaDemux/549 -> adaBCre/549  "Suspension:base_velocity:R1"
  adaDemux/550 -> adaBCre/550  "Suspension:base_velocity:R2"
  adaDemux/551 -> adaBCre/551  "Suspension:Inst_Stiff_Deflection:front_left"
  adaDemux/552 -> adaBCre/552  "Suspension:Inst_Stiff_Deflection:front_right"
  adaDemux/553 -> adaBCre/553  "Suspension:Inst_Stiff_Deflection:rear_left"
  adaDemux/554 -> adaBCre/554  "Suspension:Inst_Stiff_Deflection:rear_right"
  adaDemux/555 -> adaBCre/555  "Suspension:Inst_Stiff_Force:front_left"
  adaDemux/556 -> adaBCre/556  "Suspension:Inst_Stiff_Force:front_right"
  adaDemux/557 -> adaBCre/557  "Suspension:Inst_Stiff_Force:rear_left"
  adaDemux/558 -> adaBCre/558  "Suspension:Inst_Stiff_Force:rear_right"
  adaDemux/559 -> adaBCre/559  "Suspension:Jounce:L1"
  adaDemux/560 -> adaBCre/560  "Suspension:Jounce:L2"
  adaDemux/561 -> adaBCre/561  "Suspension:Jounce:R1"
  adaDemux/562 -> adaBCre/562  "Suspension:Jounce:R2"
  adaDemux/563 -> adaBCre/563  "Suspension:Jounce_Acceleration:L1"
  adaDemux/564 -> adaBCre/564  "Suspension:Jounce_Acceleration:L2"
  adaDemux/565 -> adaBCre/565  "Suspension:Jounce_Acceleration:R1"
  adaDemux/566 -> adaBCre/566  "Suspension:Jounce_Acceleration:R2"
  adaDemux/567 -> adaBCre/567  "Suspension:Jounce_Rate:L1"
  adaDemux/568 -> adaBCre/568  "Suspension:Jounce_Rate:L2"
  adaDemux/569 -> adaBCre/569  "Suspension:Jounce_Rate:R1"
  adaDemux/570 -> adaBCre/570  "Suspension:Jounce_Rate:R2"
  adaDemux/571 -> adaBCre/571  "Suspension:Kingpin_Moment:SUSP1"
  adaDemux/572 -> adaBCre/572  "Suspension:Roll:SUSP1"
  adaDemux/573 -> adaBCre/573  "Suspension:Roll:SUSP2"
  adaDemux/574 -> adaBCre/574  "Suspension:Roll_Center_Height:front"
  adaDemux/575 -> adaBCre/575  "Suspension:Roll_Center_Height:rear"
  adaDemux/576 -> adaBCre/576  "Suspension:Roll_Center_Lateral_Displacement:front"
  adaDemux/577 -> adaBCre/577  "Suspension:Roll_Center_Lateral_Displacement:rear"
  adaDemux/578 -> adaBCre/578  "Suspension:Steering_Instant_Axis_Rotation:L1"
  adaDemux/579 -> adaBCre/579  "Suspension:Steering_Instant_Axis_Rotation:R1"
  adaDemux/580 -> adaBCre/580  "System:Angular_Acceleration_Norm"
  adaDemux/581 -> adaBCre/581  "System:Angular_Speed_Norm"
  adaDemux/582 -> adaBCre/582  "System:Testrig_MMM_Fx"
  adaDemux/583 -> adaBCre/583  "System:Testrig_MMM_Fy"
  adaDemux/584 -> adaBCre/584  "System:Testrig_MMM_Mz"
  adaDemux/585 -> adaBCre/585  "System:Testrig_MMM_xd"
  adaDemux/586 -> adaBCre/586  "System:Testrig_MMM_xi"
  adaDemux/587 -> adaBCre/587  "System:Testrig_MMM_xp"
  adaDemux/588 -> adaBCre/588  "System:Testrig_MMM_yawd"
  adaDemux/589 -> adaBCre/589  "System:Testrig_MMM_yawi"
  adaDemux/590 -> adaBCre/590  "System:Testrig_MMM_yawp"
  adaDemux/591 -> adaBCre/591  "System:Testrig_MMM_yd"
  adaDemux/592 -> adaBCre/592  "System:Testrig_MMM_yi"
  adaDemux/593 -> adaBCre/593  "System:Testrig_MMM_yp"
  adaDemux/594 -> adaBCre/594  "System:Time"
  adaDemux/595 -> adaBCre/595  "System:Translational_Acceleration_Norm"
  adaDemux/596 -> adaBCre/596  "System:Translational_Speed_Norm"
  adaDemux/597 -> adaBCre/597  "System:Solver_Status"
  adaDemux/598 -> adaBCre/598  "System_Mass_Center:Global_Ax"
  adaDemux/599 -> adaBCre/599  "System_Mass_Center:Global_Ay"
  adaDemux/600 -> adaBCre/600  "System_Mass_Center:Global_Az"
  adaDemux/601 -> adaBCre/601  "System_Mass_Center:Global_Vx"
  adaDemux/602 -> adaBCre/602  "System_Mass_Center:Global_Vy"
  adaDemux/603 -> adaBCre/603  "System_Mass_Center:Global_Vz"
  adaDemux/604 -> adaBCre/604  "System_Mass_Center:Global_X"
  adaDemux/605 -> adaBCre/605  "System_Mass_Center:Global_Y"
  adaDemux/606 -> adaBCre/606  "System_Mass_Center:Global_Z"
  adaDemux/607 -> adaBCre/607  "System_Mass_Center:Normal_Acceleration"
  adaDemux/608 -> adaBCre/608  "System_Mass_Center:Path_Curvature"
  adaDemux/609 -> adaBCre/609  "System_Mass_Center:Speed"
  adaDemux/610 -> adaBCre/610  "System_Mass_Center:Tangential_Acceleration"
  adaDemux/611 -> adaBCre/611  "til_wheel_tire_forces:aligning_torque_front"
  adaDemux/612 -> adaBCre/612  "til_wheel_tire_forces:aligning_torque_rear"
  adaDemux/613 -> adaBCre/613  "til_wheel_tire_forces:aligning_torque_twin_rear"
  adaDemux/614 -> adaBCre/614  "til_wheel_tire_forces:lateral_front"
  adaDemux/615 -> adaBCre/615  "til_wheel_tire_forces:lateral_rear"
  adaDemux/616 -> adaBCre/616  "til_wheel_tire_forces:lateral_twin_rear"
  adaDemux/617 -> adaBCre/617  "til_wheel_tire_forces:longitudinal_front"
  adaDemux/618 -> adaBCre/618  "til_wheel_tire_forces:longitudinal_rear"
  adaDemux/619 -> adaBCre/619  "til_wheel_tire_forces:longitudinal_twin_rear"
  adaDemux/620 -> adaBCre/620  "til_wheel_tire_forces:normal_front"
  adaDemux/621 -> adaBCre/621  "til_wheel_tire_forces:normal_rear"
  adaDemux/622 -> adaBCre/622  "til_wheel_tire_forces:normal_twin_rear"
  adaDemux/623 -> adaBCre/623  "til_wheel_tire_forces:overturning_moment_front"
  adaDemux/624 -> adaBCre/624  "til_wheel_tire_forces:overturning_moment_rear"
  adaDemux/625 -> adaBCre/625  "til_wheel_tire_forces:overturning_moment_twin_rear"
  adaDemux/626 -> adaBCre/626  "til_wheel_tire_forces:rolling_resistance_front"
  adaDemux/627 -> adaBCre/627  "til_wheel_tire_forces:rolling_resistance_rear"
  adaDemux/628 -> adaBCre/628  "til_wheel_tire_forces:rolling_resistance_twin_rear"
  adaDemux/629 -> adaBCre/629  "til_wheel_tire_kinematics:inclination_angle_front"
  adaDemux/630 -> adaBCre/630  "til_wheel_tire_kinematics:inclination_angle_rear"
  adaDemux/631 -> adaBCre/631  "til_wheel_tire_kinematics:inclination_angle_twin_rear"
  adaDemux/632 -> adaBCre/632  "til_wheel_tire_kinematics:lateral_slip_front"
  adaDemux/633 -> adaBCre/633  "til_wheel_tire_kinematics:lateral_slip_rear"
  adaDemux/634 -> adaBCre/634  "til_wheel_tire_kinematics:lateral_slip_twin_rear"
  adaDemux/635 -> adaBCre/635  "til_wheel_tire_kinematics:longitudinal_slip_front"
  adaDemux/636 -> adaBCre/636  "til_wheel_tire_kinematics:longitudinal_slip_rear"
  adaDemux/637 -> adaBCre/637  "til_wheel_tire_kinematics:longitudinal_slip_twin_rear"
  adaDemux/638 -> adaBCre/638  "til_wheel_tire_rolling_states:omega_actual_front"
  adaDemux/639 -> adaBCre/639  "til_wheel_tire_rolling_states:omega_actual_rear"
  adaDemux/640 -> adaBCre/640  "til_wheel_tire_rolling_states:omega_actual_twin_rear"
  adaDemux/641 -> adaBCre/641  "til_wheel_tire_rolling_states:omega_free_front"
  adaDemux/642 -> adaBCre/642  "til_wheel_tire_rolling_states:omega_free_rear"
  adaDemux/643 -> adaBCre/643  "til_wheel_tire_rolling_states:omega_free_twin_rear"
  adaDemux/644 -> adaBCre/644  "til_wheel_tire_rolling_states:rolling_radius_front"
  adaDemux/645 -> adaBCre/645  "til_wheel_tire_rolling_states:rolling_radius_rear"
  adaDemux/646 -> adaBCre/646  "til_wheel_tire_rolling_states:rolling_radius_twin_rear"
  adaDemux/647 -> adaBCre/647  "Tire:Actual_Tread_Speed:L1"
  adaDemux/648 -> adaBCre/648  "Tire:Actual_Tread_Speed:L2"
  adaDemux/649 -> adaBCre/649  "Tire:Actual_Tread_Speed:R1"
  adaDemux/650 -> adaBCre/650  "Tire:Actual_Tread_Speed:R2"
  adaDemux/651 -> adaBCre/651  "Tire:Contact_Patch_Global_X:L1"
  adaDemux/652 -> adaBCre/652  "Tire:Contact_Patch_Global_X:L2"
  adaDemux/653 -> adaBCre/653  "Tire:Contact_Patch_Global_X:R1"
  adaDemux/654 -> adaBCre/654  "Tire:Contact_Patch_Global_X:R2"
  adaDemux/655 -> adaBCre/655  "Tire:Contact_Patch_Global_Y:L1"
  adaDemux/656 -> adaBCre/656  "Tire:Contact_Patch_Global_Y:L2"
  adaDemux/657 -> adaBCre/657  "Tire:Contact_Patch_Global_Y:R1"
  adaDemux/658 -> adaBCre/658  "Tire:Contact_Patch_Global_Y:R2"
  adaDemux/659 -> adaBCre/659  "Tire:Contact_Patch_Global_Z:L1"
  adaDemux/660 -> adaBCre/660  "Tire:Contact_Patch_Global_Z:L2"
  adaDemux/661 -> adaBCre/661  "Tire:Contact_Patch_Global_Z:R1"
  adaDemux/662 -> adaBCre/662  "Tire:Contact_Patch_Global_Z:R2"
  adaDemux/663 -> adaBCre/663  "Tire:Contact_Patch_Normal_X:L1"
  adaDemux/664 -> adaBCre/664  "Tire:Contact_Patch_Normal_X:L2"
  adaDemux/665 -> adaBCre/665  "Tire:Contact_Patch_Normal_X:R1"
  adaDemux/666 -> adaBCre/666  "Tire:Contact_Patch_Normal_X:R2"
  adaDemux/667 -> adaBCre/667  "Tire:Contact_Patch_Normal_Y:L1"
  adaDemux/668 -> adaBCre/668  "Tire:Contact_Patch_Normal_Y:L2"
  adaDemux/669 -> adaBCre/669  "Tire:Contact_Patch_Normal_Y:R1"
  adaDemux/670 -> adaBCre/670  "Tire:Contact_Patch_Normal_Y:R2"
  adaDemux/671 -> adaBCre/671  "Tire:Contact_Patch_Normal_Z:L1"
  adaDemux/672 -> adaBCre/672  "Tire:Contact_Patch_Normal_Z:L2"
  adaDemux/673 -> adaBCre/673  "Tire:Contact_Patch_Normal_Z:R1"
  adaDemux/674 -> adaBCre/674  "Tire:Contact_Patch_Normal_Z:R2"
  adaDemux/675 -> adaBCre/675  "Tire:Effective_Closing_Speed:L1"
  adaDemux/676 -> adaBCre/676  "Tire:Effective_Closing_Speed:L2"
  adaDemux/677 -> adaBCre/677  "Tire:Effective_Closing_Speed:R1"
  adaDemux/678 -> adaBCre/678  "Tire:Effective_Closing_Speed:R2"
  adaDemux/679 -> adaBCre/679  "Tire:Effective_Penetration:L1"
  adaDemux/680 -> adaBCre/680  "Tire:Effective_Penetration:L2"
  adaDemux/681 -> adaBCre/681  "Tire:Effective_Penetration:R1"
  adaDemux/682 -> adaBCre/682  "Tire:Effective_Penetration:R2"
  adaDemux/683 -> adaBCre/683  "Tire:Effective_Rolling_Radius:L1"
  adaDemux/684 -> adaBCre/684  "Tire:Effective_Rolling_Radius:L2"
  adaDemux/685 -> adaBCre/685  "Tire:Effective_Rolling_Radius:R1"
  adaDemux/686 -> adaBCre/686  "Tire:Effective_Rolling_Radius:R2"
  adaDemux/687 -> adaBCre/687  "Tire:Equivalent_Tread_Speed:L1"
  adaDemux/688 -> adaBCre/688  "Tire:Equivalent_Tread_Speed:L2"
  adaDemux/689 -> adaBCre/689  "Tire:Equivalent_Tread_Speed:R1"
  adaDemux/690 -> adaBCre/690  "Tire:Equivalent_Tread_Speed:R2"
  adaDemux/691 -> adaBCre/691  "Tire:External_Friction_Scale_Factor:L1"
  adaDemux/692 -> adaBCre/692  "Tire:External_Friction_Scale_Factor:L2"
  adaDemux/693 -> adaBCre/693  "Tire:External_Friction_Scale_Factor:R1"
  adaDemux/694 -> adaBCre/694  "Tire:External_Friction_Scale_Factor:R2"
  adaDemux/695 -> adaBCre/695  "Tire:Ground_Surface_Contact_Patch_Vx:L1"
  adaDemux/696 -> adaBCre/696  "Tire:Ground_Surface_Contact_Patch_Vx:L2"
  adaDemux/697 -> adaBCre/697  "Tire:Ground_Surface_Contact_Patch_Vx:R1"
  adaDemux/698 -> adaBCre/698  "Tire:Ground_Surface_Contact_Patch_Vx:R2"
  adaDemux/699 -> adaBCre/699  "Tire:Ground_Surface_Contact_Patch_Vy:L1"
  adaDemux/700 -> adaBCre/700  "Tire:Ground_Surface_Contact_Patch_Vy:L2"
  adaDemux/701 -> adaBCre/701  "Tire:Ground_Surface_Contact_Patch_Vy:R1"
  adaDemux/702 -> adaBCre/702  "Tire:Ground_Surface_Contact_Patch_Vy:R2"
  adaDemux/703 -> adaBCre/703  "Tire:Ground_Surface_Force_X:L1"
  adaDemux/704 -> adaBCre/704  "Tire:Ground_Surface_Force_X:L2"
  adaDemux/705 -> adaBCre/705  "Tire:Ground_Surface_Force_X:R1"
  adaDemux/706 -> adaBCre/706  "Tire:Ground_Surface_Force_X:R2"
  adaDemux/707 -> adaBCre/707  "Tire:Ground_Surface_Force_Y:L1"
  adaDemux/708 -> adaBCre/708  "Tire:Ground_Surface_Force_Y:L2"
  adaDemux/709 -> adaBCre/709  "Tire:Ground_Surface_Force_Y:R1"
  adaDemux/710 -> adaBCre/710  "Tire:Ground_Surface_Force_Y:R2"
  adaDemux/711 -> adaBCre/711  "Tire:Ground_Surface_Force_Z:L1"
  adaDemux/712 -> adaBCre/712  "Tire:Ground_Surface_Force_Z:L2"
  adaDemux/713 -> adaBCre/713  "Tire:Ground_Surface_Force_Z:R1"
  adaDemux/714 -> adaBCre/714  "Tire:Ground_Surface_Force_Z:R2"
  adaDemux/715 -> adaBCre/715  "Tire:Ground_Surface_Gyroscopic_Moment:L1"
  adaDemux/716 -> adaBCre/716  "Tire:Ground_Surface_Gyroscopic_Moment:L2"
  adaDemux/717 -> adaBCre/717  "Tire:Ground_Surface_Gyroscopic_Moment:R1"
  adaDemux/718 -> adaBCre/718  "Tire:Ground_Surface_Gyroscopic_Moment:R2"
  adaDemux/719 -> adaBCre/719  "Tire:Ground_Surface_Kappa_Fy:L1"
  adaDemux/720 -> adaBCre/720  "Tire:Ground_Surface_Kappa_Fy:L2"
  adaDemux/721 -> adaBCre/721  "Tire:Ground_Surface_Kappa_Fy:R1"
  adaDemux/722 -> adaBCre/722  "Tire:Ground_Surface_Kappa_Fy:R2"
  adaDemux/723 -> adaBCre/723  "Tire:Ground_Surface_Moment_X:L1"
  adaDemux/724 -> adaBCre/724  "Tire:Ground_Surface_Moment_X:L2"
  adaDemux/725 -> adaBCre/725  "Tire:Ground_Surface_Moment_X:R1"
  adaDemux/726 -> adaBCre/726  "Tire:Ground_Surface_Moment_X:R2"
  adaDemux/727 -> adaBCre/727  "Tire:Ground_Surface_Moment_Y:L1"
  adaDemux/728 -> adaBCre/728  "Tire:Ground_Surface_Moment_Y:L2"
  adaDemux/729 -> adaBCre/729  "Tire:Ground_Surface_Moment_Y:R1"
  adaDemux/730 -> adaBCre/730  "Tire:Ground_Surface_Moment_Y:R2"
  adaDemux/731 -> adaBCre/731  "Tire:Ground_Surface_Moment_Z:L1"
  adaDemux/732 -> adaBCre/732  "Tire:Ground_Surface_Moment_Z:L2"
  adaDemux/733 -> adaBCre/733  "Tire:Ground_Surface_Moment_Z:R1"
  adaDemux/734 -> adaBCre/734  "Tire:Ground_Surface_Moment_Z:R2"
  adaDemux/735 -> adaBCre/735  "Tire:Ground_Surface_Peak_Friction_X:L1"
  adaDemux/736 -> adaBCre/736  "Tire:Ground_Surface_Peak_Friction_X:L2"
  adaDemux/737 -> adaBCre/737  "Tire:Ground_Surface_Peak_Friction_X:R1"
  adaDemux/738 -> adaBCre/738  "Tire:Ground_Surface_Peak_Friction_X:R2"
  adaDemux/739 -> adaBCre/739  "Tire:Ground_Surface_Peak_Friction_Y:L1"
  adaDemux/740 -> adaBCre/740  "Tire:Ground_Surface_Peak_Friction_Y:L2"
  adaDemux/741 -> adaBCre/741  "Tire:Ground_Surface_Peak_Friction_Y:R1"
  adaDemux/742 -> adaBCre/742  "Tire:Ground_Surface_Peak_Friction_Y:R2"
  adaDemux/743 -> adaBCre/743  "Tire:Ground_Surface_Residual_Torque:L1"
  adaDemux/744 -> adaBCre/744  "Tire:Ground_Surface_Residual_Torque:L2"
  adaDemux/745 -> adaBCre/745  "Tire:Ground_Surface_Residual_Torque:R1"
  adaDemux/746 -> adaBCre/746  "Tire:Ground_Surface_Residual_Torque:R2"
  adaDemux/747 -> adaBCre/747  "Tire:Hub_Carrier_Force_Global_X:L1"
  adaDemux/748 -> adaBCre/748  "Tire:Hub_Carrier_Force_Global_X:L2"
  adaDemux/749 -> adaBCre/749  "Tire:Hub_Carrier_Force_Global_X:R1"
  adaDemux/750 -> adaBCre/750  "Tire:Hub_Carrier_Force_Global_X:R2"
  adaDemux/751 -> adaBCre/751  "Tire:Hub_Carrier_Force_Global_Y:L1"
  adaDemux/752 -> adaBCre/752  "Tire:Hub_Carrier_Force_Global_Y:L2"
  adaDemux/753 -> adaBCre/753  "Tire:Hub_Carrier_Force_Global_Y:R1"
  adaDemux/754 -> adaBCre/754  "Tire:Hub_Carrier_Force_Global_Y:R2"
  adaDemux/755 -> adaBCre/755  "Tire:Hub_Carrier_Force_Global_Z:L1"
  adaDemux/756 -> adaBCre/756  "Tire:Hub_Carrier_Force_Global_Z:L2"
  adaDemux/757 -> adaBCre/757  "Tire:Hub_Carrier_Force_Global_Z:R1"
  adaDemux/758 -> adaBCre/758  "Tire:Hub_Carrier_Force_Global_Z:R2"
  adaDemux/759 -> adaBCre/759  "Tire:Hub_Carrier_Force_Local_X:L1"
  adaDemux/760 -> adaBCre/760  "Tire:Hub_Carrier_Force_Local_X:L2"
  adaDemux/761 -> adaBCre/761  "Tire:Hub_Carrier_Force_Local_X:R1"
  adaDemux/762 -> adaBCre/762  "Tire:Hub_Carrier_Force_Local_X:R2"
  adaDemux/763 -> adaBCre/763  "Tire:Hub_Carrier_Force_Local_Y:L1"
  adaDemux/764 -> adaBCre/764  "Tire:Hub_Carrier_Force_Local_Y:L2"
  adaDemux/765 -> adaBCre/765  "Tire:Hub_Carrier_Force_Local_Y:R1"
  adaDemux/766 -> adaBCre/766  "Tire:Hub_Carrier_Force_Local_Y:R2"
  adaDemux/767 -> adaBCre/767  "Tire:Hub_Carrier_Force_Local_Z:L1"
  adaDemux/768 -> adaBCre/768  "Tire:Hub_Carrier_Force_Local_Z:L2"
  adaDemux/769 -> adaBCre/769  "Tire:Hub_Carrier_Force_Local_Z:R1"
  adaDemux/770 -> adaBCre/770  "Tire:Hub_Carrier_Force_Local_Z:R2"
  adaDemux/771 -> adaBCre/771  "Tire:Hub_Carrier_Moment_Global_X:L1"
  adaDemux/772 -> adaBCre/772  "Tire:Hub_Carrier_Moment_Global_X:L2"
  adaDemux/773 -> adaBCre/773  "Tire:Hub_Carrier_Moment_Global_X:R1"
  adaDemux/774 -> adaBCre/774  "Tire:Hub_Carrier_Moment_Global_X:R2"
  adaDemux/775 -> adaBCre/775  "Tire:Hub_Carrier_Moment_Global_Y:L1"
  adaDemux/776 -> adaBCre/776  "Tire:Hub_Carrier_Moment_Global_Y:L2"
  adaDemux/777 -> adaBCre/777  "Tire:Hub_Carrier_Moment_Global_Y:R1"
  adaDemux/778 -> adaBCre/778  "Tire:Hub_Carrier_Moment_Global_Y:R2"
  adaDemux/779 -> adaBCre/779  "Tire:Hub_Carrier_Moment_Global_Z:L1"
  adaDemux/780 -> adaBCre/780  "Tire:Hub_Carrier_Moment_Global_Z:L2"
  adaDemux/781 -> adaBCre/781  "Tire:Hub_Carrier_Moment_Global_Z:R1"
  adaDemux/782 -> adaBCre/782  "Tire:Hub_Carrier_Moment_Global_Z:R2"
  adaDemux/783 -> adaBCre/783  "Tire:Hub_Carrier_Moment_Local_X:L1"
  adaDemux/784 -> adaBCre/784  "Tire:Hub_Carrier_Moment_Local_X:L2"
  adaDemux/785 -> adaBCre/785  "Tire:Hub_Carrier_Moment_Local_X:R1"
  adaDemux/786 -> adaBCre/786  "Tire:Hub_Carrier_Moment_Local_X:R2"
  adaDemux/787 -> adaBCre/787  "Tire:Hub_Carrier_Moment_Local_Y:L1"
  adaDemux/788 -> adaBCre/788  "Tire:Hub_Carrier_Moment_Local_Y:L2"
  adaDemux/789 -> adaBCre/789  "Tire:Hub_Carrier_Moment_Local_Y:R1"
  adaDemux/790 -> adaBCre/790  "Tire:Hub_Carrier_Moment_Local_Y:R2"
  adaDemux/791 -> adaBCre/791  "Tire:Hub_Carrier_Moment_Local_Z:L1"
  adaDemux/792 -> adaBCre/792  "Tire:Hub_Carrier_Moment_Local_Z:L2"
  adaDemux/793 -> adaBCre/793  "Tire:Hub_Carrier_Moment_Local_Z:R1"
  adaDemux/794 -> adaBCre/794  "Tire:Hub_Carrier_Moment_Local_Z:R2"
  adaDemux/795 -> adaBCre/795  "Tire:Lateral_Relaxation_Length:L1"
  adaDemux/796 -> adaBCre/796  "Tire:Lateral_Relaxation_Length:L2"
  adaDemux/797 -> adaBCre/797  "Tire:Lateral_Relaxation_Length:R1"
  adaDemux/798 -> adaBCre/798  "Tire:Lateral_Relaxation_Length:R2"
  adaDemux/799 -> adaBCre/799  "Tire:Lateral_Slip_Without_Lag:L1"
  adaDemux/800 -> adaBCre/800  "Tire:Lateral_Slip_Without_Lag:L2"
  adaDemux/801 -> adaBCre/801  "Tire:Lateral_Slip_Without_Lag:R1"
  adaDemux/802 -> adaBCre/802  "Tire:Lateral_Slip_Without_Lag:R2"
  adaDemux/803 -> adaBCre/803  "Tire:Lateral_Slip_With_Lag:L1"
  adaDemux/804 -> adaBCre/804  "Tire:Lateral_Slip_With_Lag:L2"
  adaDemux/805 -> adaBCre/805  "Tire:Lateral_Slip_With_Lag:R1"
  adaDemux/806 -> adaBCre/806  "Tire:Lateral_Slip_With_Lag:R2"
  adaDemux/807 -> adaBCre/807  "Tire:Loaded_Radius:L1"
  adaDemux/808 -> adaBCre/808  "Tire:Loaded_Radius:L2"
  adaDemux/809 -> adaBCre/809  "Tire:Loaded_Radius:R1"
  adaDemux/810 -> adaBCre/810  "Tire:Loaded_Radius:R2"
  adaDemux/811 -> adaBCre/811  "Tire:Longitudinal_Relaxation_Length:L1"
  adaDemux/812 -> adaBCre/812  "Tire:Longitudinal_Relaxation_Length:L2"
  adaDemux/813 -> adaBCre/813  "Tire:Longitudinal_Relaxation_Length:R1"
  adaDemux/814 -> adaBCre/814  "Tire:Longitudinal_Relaxation_Length:R2"
  adaDemux/815 -> adaBCre/815  "Tire:Longitudinal_Slip_Without_Lag:L1"
  adaDemux/816 -> adaBCre/816  "Tire:Longitudinal_Slip_Without_Lag:L2"
  adaDemux/817 -> adaBCre/817  "Tire:Longitudinal_Slip_Without_Lag:R1"
  adaDemux/818 -> adaBCre/818  "Tire:Longitudinal_Slip_Without_Lag:R2"
  adaDemux/819 -> adaBCre/819  "Tire:Longitudinal_Slip_With_Lag:L1"
  adaDemux/820 -> adaBCre/820  "Tire:Longitudinal_Slip_With_Lag:L2"
  adaDemux/821 -> adaBCre/821  "Tire:Longitudinal_Slip_With_Lag:R1"
  adaDemux/822 -> adaBCre/822  "Tire:Longitudinal_Slip_With_Lag:R2"
  adaDemux/823 -> adaBCre/823  "Tire:Moment_Arm_Of_Fx:L1"
  adaDemux/824 -> adaBCre/824  "Tire:Moment_Arm_Of_Fx:L2"
  adaDemux/825 -> adaBCre/825  "Tire:Moment_Arm_Of_Fx:R1"
  adaDemux/826 -> adaBCre/826  "Tire:Moment_Arm_Of_Fx:R2"
  adaDemux/827 -> adaBCre/827  "Tire:Pneumatic_Trail:L1"
  adaDemux/828 -> adaBCre/828  "Tire:Pneumatic_Trail:L2"
  adaDemux/829 -> adaBCre/829  "Tire:Pneumatic_Trail:R1"
  adaDemux/830 -> adaBCre/830  "Tire:Pneumatic_Trail:R2"
  adaDemux/831 -> adaBCre/831  "Tire:Pressure:L1"
  adaDemux/832 -> adaBCre/832  "Tire:Pressure:L2"
  adaDemux/833 -> adaBCre/833  "Tire:Pressure:R1"
  adaDemux/834 -> adaBCre/834  "Tire:Pressure:R2"
  adaDemux/835 -> adaBCre/835  "Tire:Road_friction:L1"
  adaDemux/836 -> adaBCre/836  "Tire:Road_friction:L2"
  adaDemux/837 -> adaBCre/837  "Tire:Road_friction:R1"
  adaDemux/838 -> adaBCre/838  "Tire:Road_friction:R2"
  adaDemux/839 -> adaBCre/839  "Tire:Temperature_1:L1"
  adaDemux/840 -> adaBCre/840  "Tire:Temperature_1:L2"
  adaDemux/841 -> adaBCre/841  "Tire:Temperature_1:R1"
  adaDemux/842 -> adaBCre/842  "Tire:Temperature_1:R2"
  adaDemux/843 -> adaBCre/843  "Tire:Temperature_2:L1"
  adaDemux/844 -> adaBCre/844  "Tire:Temperature_2:L2"
  adaDemux/845 -> adaBCre/845  "Tire:Temperature_2:R1"
  adaDemux/846 -> adaBCre/846  "Tire:Temperature_2:R2"
  adaDemux/847 -> adaBCre/847  "Tire:Temperature_3:L1"
  adaDemux/848 -> adaBCre/848  "Tire:Temperature_3:L2"
  adaDemux/849 -> adaBCre/849  "Tire:Temperature_3:R1"
  adaDemux/850 -> adaBCre/850  "Tire:Temperature_3:R2"
  adaDemux/851 -> adaBCre/851  "Tire:Temperature_4:L1"
  adaDemux/852 -> adaBCre/852  "Tire:Temperature_4:L2"
  adaDemux/853 -> adaBCre/853  "Tire:Temperature_4:R1"
  adaDemux/854 -> adaBCre/854  "Tire:Temperature_4:R2"
  adaDemux/855 -> adaBCre/855  "Tire:User_Input_Contact_Patch_Global_Z_Perturbation:L1"
  adaDemux/856 -> adaBCre/856  "Tire:User_Input_Contact_Patch_Global_Z_Perturbation:L2"
  adaDemux/857 -> adaBCre/857  "Tire:User_Input_Contact_Patch_Global_Z_Perturbation:R1"
  adaDemux/858 -> adaBCre/858  "Tire:User_Input_Contact_Patch_Global_Z_Perturbation:R2"
  adaDemux/859 -> adaBCre/859  "Tire:Wear:L1"
  adaDemux/860 -> adaBCre/860  "Tire:Wear:L2"
  adaDemux/861 -> adaBCre/861  "Tire:Wear:R1"
  adaDemux/862 -> adaBCre/862  "Tire:Wear:R2"
  adaDemux/863 -> adaBCre/863  "tir_wheel_tire_forces:aligning_torque_front"
  adaDemux/864 -> adaBCre/864  "tir_wheel_tire_forces:aligning_torque_rear"
  adaDemux/865 -> adaBCre/865  "tir_wheel_tire_forces:aligning_torque_twin_rear"
  adaDemux/866 -> adaBCre/866  "tir_wheel_tire_forces:lateral_front"
  adaDemux/867 -> adaBCre/867  "tir_wheel_tire_forces:lateral_rear"
  adaDemux/868 -> adaBCre/868  "tir_wheel_tire_forces:lateral_twin_rear"
  adaDemux/869 -> adaBCre/869  "tir_wheel_tire_forces:longitudinal_front"
  adaDemux/870 -> adaBCre/870  "tir_wheel_tire_forces:longitudinal_rear"
  adaDemux/871 -> adaBCre/871  "tir_wheel_tire_forces:longitudinal_twin_rear"
  adaDemux/872 -> adaBCre/872  "tir_wheel_tire_forces:normal_front"
  adaDemux/873 -> adaBCre/873  "tir_wheel_tire_forces:normal_rear"
  adaDemux/874 -> adaBCre/874  "tir_wheel_tire_forces:normal_twin_rear"
  adaDemux/875 -> adaBCre/875  "tir_wheel_tire_forces:overturning_moment_front"
  adaDemux/876 -> adaBCre/876  "tir_wheel_tire_forces:overturning_moment_rear"
  adaDemux/877 -> adaBCre/877  "tir_wheel_tire_forces:overturning_moment_twin_rear"
  adaDemux/878 -> adaBCre/878  "tir_wheel_tire_forces:rolling_resistance_front"
  adaDemux/879 -> adaBCre/879  "tir_wheel_tire_forces:rolling_resistance_rear"
  adaDemux/880 -> adaBCre/880  "tir_wheel_tire_forces:rolling_resistance_twin_rear"
  adaDemux/881 -> adaBCre/881  "tir_wheel_tire_kinematics:inclination_angle_front"
  adaDemux/882 -> adaBCre/882  "tir_wheel_tire_kinematics:inclination_angle_rear"
  adaDemux/883 -> adaBCre/883  "tir_wheel_tire_kinematics:inclination_angle_twin_rear"
  adaDemux/884 -> adaBCre/884  "tir_wheel_tire_kinematics:lateral_slip_front"
  adaDemux/885 -> adaBCre/885  "tir_wheel_tire_kinematics:lateral_slip_rear"
  adaDemux/886 -> adaBCre/886  "tir_wheel_tire_kinematics:lateral_slip_twin_rear"
  adaDemux/887 -> adaBCre/887  "tir_wheel_tire_kinematics:longitudinal_slip_front"
  adaDemux/888 -> adaBCre/888  "tir_wheel_tire_kinematics:longitudinal_slip_rear"
  adaDemux/889 -> adaBCre/889  "tir_wheel_tire_kinematics:longitudinal_slip_twin_rear"
  adaDemux/890 -> adaBCre/890  "tir_wheel_tire_rolling_states:omega_actual_front"
  adaDemux/891 -> adaBCre/891  "tir_wheel_tire_rolling_states:omega_actual_rear"
  adaDemux/892 -> adaBCre/892  "tir_wheel_tire_rolling_states:omega_actual_twin_rear"
  adaDemux/893 -> adaBCre/893  "tir_wheel_tire_rolling_states:omega_free_front"
  adaDemux/894 -> adaBCre/894  "tir_wheel_tire_rolling_states:omega_free_rear"
  adaDemux/895 -> adaBCre/895  "tir_wheel_tire_rolling_states:omega_free_twin_rear"
  adaDemux/896 -> adaBCre/896  "tir_wheel_tire_rolling_states:rolling_radius_front"
  adaDemux/897 -> adaBCre/897  "tir_wheel_tire_rolling_states:rolling_radius_rear"
  adaDemux/898 -> adaBCre/898  "tir_wheel_tire_rolling_states:rolling_radius_twin_rear"
  adaDemux/899 -> adaBCre/899  "torque_converter:capacity_factor"
  adaDemux/900 -> adaBCre/900  "torque_converter:efficiency"
  adaDemux/901 -> adaBCre/901  "torque_converter:gearbox_inputshaft_alpha"
  adaDemux/902 -> adaBCre/902  "torque_converter:gearbox_inputshaft_angle"
  adaDemux/903 -> adaBCre/903  "torque_converter:gearbox_inputshaft_omega"
  adaDemux/904 -> adaBCre/904  "torque_converter:inputplate_torque"
  adaDemux/905 -> adaBCre/905  "torque_converter:speed_ratio"
  adaDemux/906 -> adaBCre/906  "torque_converter:torque"
  adaDemux/907 -> adaBCre/907  "torque_converter:torque_ratio"
  adaDemux/908 -> adaBCre/908  "transmission:automatic_gearbox_shifting_mode"
  adaDemux/909 -> adaBCre/909  "transmission:clutch_outputplate_torque"
  adaDemux/910 -> adaBCre/910  "transmission:diff_central_inputshaft_alpha"
  adaDemux/911 -> adaBCre/911  "transmission:diff_central_inputshaft_angle"
  adaDemux/912 -> adaBCre/912  "transmission:diff_central_inputshaft_omega"
  adaDemux/913 -> adaBCre/913  "transmission:gear"
  adaDemux/914 -> adaBCre/914  "transmission:input_rpm"
  adaDemux/915 -> adaBCre/915  "transmission:output_rpm"
  adaDemux/916 -> adaBCre/916  "transmission:ratio"
  adaDemux/917 -> adaBCre/917  "transmission:torque"
  adaDemux/918 -> adaBCre/918  "transmission:manual_shifting_activity"
  adaDemux/919 -> adaBCre/919  "ues_third_spring_data:displacement_front"
  adaDemux/920 -> adaBCre/920  "ues_third_spring_data:displacement_rear"
  adaDemux/921 -> adaBCre/921  "ues_third_spring_data:force_front"
  adaDemux/922 -> adaBCre/922  "ues_third_spring_data:force_rear"
  adaDemux/923 -> adaBCre/923  "ues_third_spring_data:velocity_front"
  adaDemux/924 -> adaBCre/924  "ues_third_spring_data:velocity_rear"
  adaDemux/925 -> adaBCre/925  "upright_accelerometer:Z_left_front"
  adaDemux/926 -> adaBCre/926  "upright_accelerometer:Z_left_rear"
  adaDemux/927 -> adaBCre/927  "upright_accelerometer:Z_right_front"
  adaDemux/928 -> adaBCre/928  "upright_accelerometer:Z_right_rear"
  adaDemux/929 -> adaBCre/929  "Vehicle:Body_Fixed_Alpha_X"
  adaDemux/930 -> adaBCre/930  "Vehicle:Body_Fixed_Alpha_Y"
  adaDemux/931 -> adaBCre/931  "Vehicle:Body_Fixed_Alpha_Z"
  adaDemux/932 -> adaBCre/932  "Vehicle:Body_Fixed_Omega_X"
  adaDemux/933 -> adaBCre/933  "Vehicle:Body_Fixed_Omega_Y"
  adaDemux/934 -> adaBCre/934  "Vehicle:Body_Fixed_Omega_Z"
  adaDemux/935 -> adaBCre/935  "Vehicle:CM_Body_Fixed_Ax"
  adaDemux/936 -> adaBCre/936  "Vehicle:CM_Body_Fixed_Ay"
  adaDemux/937 -> adaBCre/937  "Vehicle:CM_Body_Fixed_Az"
  adaDemux/938 -> adaBCre/938  "Vehicle:CM_Body_Fixed_Vx"
  adaDemux/939 -> adaBCre/939  "Vehicle:CM_Body_Fixed_Vy"
  adaDemux/940 -> adaBCre/940  "Vehicle:CM_Body_Fixed_Vz"
  adaDemux/941 -> adaBCre/941  "Vehicle:CM_Global_And_Tracking_Az"
  adaDemux/942 -> adaBCre/942  "Vehicle:CM_Global_And_Tracking_Vz"
  adaDemux/943 -> adaBCre/943  "Vehicle:CM_Global_Ax"
  adaDemux/944 -> adaBCre/944  "Vehicle:CM_Global_Ay"
  adaDemux/945 -> adaBCre/945  "Vehicle:CM_Global_Vx"
  adaDemux/946 -> adaBCre/946  "Vehicle:CM_Global_Vy"
  adaDemux/947 -> adaBCre/947  "Vehicle:CM_Global_X"
  adaDemux/948 -> adaBCre/948  "Vehicle:CM_Global_Y"
  adaDemux/949 -> adaBCre/949  "Vehicle:CM_Global_Z"
  adaDemux/950 -> adaBCre/950  "Vehicle:CM_Tracking_Ax"
  adaDemux/951 -> adaBCre/951  "Vehicle:CM_Tracking_Ay"
  adaDemux/952 -> adaBCre/952  "Vehicle:CM_Tracking_Vx"
  adaDemux/953 -> adaBCre/953  "Vehicle:CM_Tracking_Vy"
  adaDemux/954 -> adaBCre/954  "Vehicle:cross_weight_PID"
  adaDemux/955 -> adaBCre/955  "Vehicle:Euler_Roll"
  adaDemux/956 -> adaBCre/956  "Vehicle:front_ride_height_at_center_point"
  adaDemux/957 -> adaBCre/957  "Vehicle:Global_Alpha_X"
  adaDemux/958 -> adaBCre/958  "Vehicle:Global_Alpha_Y"
  adaDemux/959 -> adaBCre/959  "Vehicle:Global_Alpha_Z"
  adaDemux/960 -> adaBCre/960  "Vehicle:Global_Omega_X"
  adaDemux/961 -> adaBCre/961  "Vehicle:Global_Omega_Y"
  adaDemux/962 -> adaBCre/962  "Vehicle:Global_Omega_Z"
  adaDemux/963 -> adaBCre/963  "Vehicle:Inclination_Roll"
  adaDemux/964 -> adaBCre/964  "Vehicle:Origin_Distance_Traveled"
  adaDemux/965 -> adaBCre/965  "Vehicle:Origin_Global_X"
  adaDemux/966 -> adaBCre/966  "Vehicle:Origin_Global_Y"
  adaDemux/967 -> adaBCre/967  "Vehicle:Origin_Global_Z"
  adaDemux/968 -> adaBCre/968  "Vehicle:Origin_Global_Z_wrt_road_mk"
  adaDemux/969 -> adaBCre/969  "Vehicle:Pitch"
  adaDemux/970 -> adaBCre/970  "Vehicle:Side_Slip_Angle"
  adaDemux/971 -> adaBCre/971  "Vehicle:Side_Slip_Angle_Rate"
  adaDemux/972 -> adaBCre/972  "Vehicle:Understeer_Gradient"
  adaDemux/973 -> adaBCre/973  "Vehicle:Understeer_Stability_Factor"
  adaDemux/974 -> adaBCre/974  "Vehicle:Yaw"
  adaDemux/975 -> adaBCre/975  "Vehicle_States:horizontal_vel_wrt_road"
  adaDemux/976 -> adaBCre/976  "Vehicle_States:lateral_acc_wrt_road"
  adaDemux/977 -> adaBCre/977  "Vehicle_States:lateral_disp"
  adaDemux/978 -> adaBCre/978  "Vehicle_States:lateral_vel_wrt_road"
  adaDemux/979 -> adaBCre/979  "Vehicle_States:longitudinal_acc_wrt_road"
  adaDemux/980 -> adaBCre/980  "Vehicle_States:longitudinal_disp"
  adaDemux/981 -> adaBCre/981  "Vehicle_States:longitudinal_vel_wrt_road"
  adaDemux/982 -> adaBCre/982  "Vehicle_States:pitch_angle"
  adaDemux/983 -> adaBCre/983  "Vehicle_States:pitch_angular_acc_wrt_road"
  adaDemux/984 -> adaBCre/984  "Vehicle_States:pitch_angular_vel_wrt_road"
  adaDemux/985 -> adaBCre/985  "Vehicle_States:roll_angle"
  adaDemux/986 -> adaBCre/986  "Vehicle_States:roll_angular_acc_wrt_road"
  adaDemux/987 -> adaBCre/987  "Vehicle_States:roll_angular_vel_wrt_road"
  adaDemux/988 -> adaBCre/988  "Vehicle_States:side_slip"
  adaDemux/989 -> adaBCre/989  "Vehicle_States:vertical_acc_wrt_road"
  adaDemux/990 -> adaBCre/990  "Vehicle_States:vertical_disp"
  adaDemux/991 -> adaBCre/991  "Vehicle_States:vertical_vel_wrt_road"
  adaDemux/992 -> adaBCre/992  "Vehicle_States:yaw_angle"
  adaDemux/993 -> adaBCre/993  "Vehicle_States:yaw_angular_acc_wrt_road"
  adaDemux/994 -> adaBCre/994  "Vehicle_States:yaw_angular_vel_wrt_road"
  adaDemux/995 -> adaBCre/995  "Wheel:Alpha:L1"
  adaDemux/996 -> adaBCre/996  "Wheel:Alpha:L2"
  adaDemux/997 -> adaBCre/997  "Wheel:Alpha:R1"
  adaDemux/998 -> adaBCre/998  "Wheel:Alpha:R2"
  adaDemux/999 -> adaBCre/999  "Wheel:Caster_Angle:left"
  adaDemux/1000 -> adaBCre/1000  "Wheel:Caster_Angle:right"
  adaDemux/1001 -> adaBCre/1001  "Wheel:Drive_Moment:L1"
  adaDemux/1002 -> adaBCre/1002  "Wheel:Drive_Moment:L2"
  adaDemux/1003 -> adaBCre/1003  "Wheel:Drive_Moment:R1"
  adaDemux/1004 -> adaBCre/1004  "Wheel:Drive_Moment:R2"
  adaDemux/1005 -> adaBCre/1005  "Wheel:Euler_Roll:L1"
  adaDemux/1006 -> adaBCre/1006  "Wheel:Euler_Roll:L2"
  adaDemux/1007 -> adaBCre/1007  "Wheel:Euler_Roll:R1"
  adaDemux/1008 -> adaBCre/1008  "Wheel:Euler_Roll:R2"
  adaDemux/1009 -> adaBCre/1009  "Wheel:Global_Omega_X:L1"
  adaDemux/1010 -> adaBCre/1010  "Wheel:Global_Omega_X:L2"
  adaDemux/1011 -> adaBCre/1011  "Wheel:Global_Omega_X:R1"
  adaDemux/1012 -> adaBCre/1012  "Wheel:Global_Omega_X:R2"
  adaDemux/1013 -> adaBCre/1013  "Wheel:Global_Omega_Y:L1"
  adaDemux/1014 -> adaBCre/1014  "Wheel:Global_Omega_Y:L2"
  adaDemux/1015 -> adaBCre/1015  "Wheel:Global_Omega_Y:R1"
  adaDemux/1016 -> adaBCre/1016  "Wheel:Global_Omega_Y:R2"
  adaDemux/1017 -> adaBCre/1017  "Wheel:Global_Omega_Z:L1"
  adaDemux/1018 -> adaBCre/1018  "Wheel:Global_Omega_Z:L2"
  adaDemux/1019 -> adaBCre/1019  "Wheel:Global_Omega_Z:R1"
  adaDemux/1020 -> adaBCre/1020  "Wheel:Global_Omega_Z:R2"
  adaDemux/1021 -> adaBCre/1021  "Wheel:Global_Vx:L1"
  adaDemux/1022 -> adaBCre/1022  "Wheel:Global_Vx:L2"
  adaDemux/1023 -> adaBCre/1023  "Wheel:Global_Vx:R1"
  adaDemux/1024 -> adaBCre/1024  "Wheel:Global_Vx:R2"
  adaDemux/1025 -> adaBCre/1025  "Wheel:Global_Vy:L1"
  adaDemux/1026 -> adaBCre/1026  "Wheel:Global_Vy:L2"
  adaDemux/1027 -> adaBCre/1027  "Wheel:Global_Vy:R1"
  adaDemux/1028 -> adaBCre/1028  "Wheel:Global_Vy:R2"
  adaDemux/1029 -> adaBCre/1029  "Wheel:Global_Vz:L1"
  adaDemux/1030 -> adaBCre/1030  "Wheel:Global_Vz:L2"
  adaDemux/1031 -> adaBCre/1031  "Wheel:Global_Vz:R1"
  adaDemux/1032 -> adaBCre/1032  "Wheel:Global_Vz:R2"
  adaDemux/1033 -> adaBCre/1033  "Wheel:Global_X:L1"
  adaDemux/1034 -> adaBCre/1034  "Wheel:Global_X:L2"
  adaDemux/1035 -> adaBCre/1035  "Wheel:Global_X:R1"
  adaDemux/1036 -> adaBCre/1036  "Wheel:Global_X:R2"
  adaDemux/1037 -> adaBCre/1037  "Wheel:Global_Y:L1"
  adaDemux/1038 -> adaBCre/1038  "Wheel:Global_Y:L2"
  adaDemux/1039 -> adaBCre/1039  "Wheel:Global_Y:R1"
  adaDemux/1040 -> adaBCre/1040  "Wheel:Global_Y:R2"
  adaDemux/1041 -> adaBCre/1041  "Wheel:Global_Z:L1"
  adaDemux/1042 -> adaBCre/1042  "Wheel:Global_Z:L2"
  adaDemux/1043 -> adaBCre/1043  "Wheel:Global_Z:R1"
  adaDemux/1044 -> adaBCre/1044  "Wheel:Global_Z:R2"
  adaDemux/1045 -> adaBCre/1045  "Wheel:Ground_Surface_Wheel_Center_Vx:L1"
  adaDemux/1046 -> adaBCre/1046  "Wheel:Ground_Surface_Wheel_Center_Vx:L2"
  adaDemux/1047 -> adaBCre/1047  "Wheel:Ground_Surface_Wheel_Center_Vx:R1"
  adaDemux/1048 -> adaBCre/1048  "Wheel:Ground_Surface_Wheel_Center_Vx:R2"
  adaDemux/1049 -> adaBCre/1049  "Wheel:Hub_Carrier_Omega_X:L1"
  adaDemux/1050 -> adaBCre/1050  "Wheel:Hub_Carrier_Omega_X:L2"
  adaDemux/1051 -> adaBCre/1051  "Wheel:Hub_Carrier_Omega_X:R1"
  adaDemux/1052 -> adaBCre/1052  "Wheel:Hub_Carrier_Omega_X:R2"
  adaDemux/1053 -> adaBCre/1053  "Wheel:Hub_Carrier_Omega_Y:L1"
  adaDemux/1054 -> adaBCre/1054  "Wheel:Hub_Carrier_Omega_Y:L2"
  adaDemux/1055 -> adaBCre/1055  "Wheel:Hub_Carrier_Omega_Y:R1"
  adaDemux/1056 -> adaBCre/1056  "Wheel:Hub_Carrier_Omega_Y:R2"
  adaDemux/1057 -> adaBCre/1057  "Wheel:Hub_Carrier_Omega_Z:L1"
  adaDemux/1058 -> adaBCre/1058  "Wheel:Hub_Carrier_Omega_Z:L2"
  adaDemux/1059 -> adaBCre/1059  "Wheel:Hub_Carrier_Omega_Z:R1"
  adaDemux/1060 -> adaBCre/1060  "Wheel:Hub_Carrier_Omega_Z:R2"
  adaDemux/1061 -> adaBCre/1061  "Wheel:Hub_Carrier_Vx:L1"
  adaDemux/1062 -> adaBCre/1062  "Wheel:Hub_Carrier_Vx:L2"
  adaDemux/1063 -> adaBCre/1063  "Wheel:Hub_Carrier_Vx:R1"
  adaDemux/1064 -> adaBCre/1064  "Wheel:Hub_Carrier_Vx:R2"
  adaDemux/1065 -> adaBCre/1065  "Wheel:Hub_Carrier_Vy:L1"
  adaDemux/1066 -> adaBCre/1066  "Wheel:Hub_Carrier_Vy:L2"
  adaDemux/1067 -> adaBCre/1067  "Wheel:Hub_Carrier_Vy:R1"
  adaDemux/1068 -> adaBCre/1068  "Wheel:Hub_Carrier_Vy:R2"
  adaDemux/1069 -> adaBCre/1069  "Wheel:Hub_Carrier_Vz:L1"
  adaDemux/1070 -> adaBCre/1070  "Wheel:Hub_Carrier_Vz:L2"
  adaDemux/1071 -> adaBCre/1071  "Wheel:Hub_Carrier_Vz:R1"
  adaDemux/1072 -> adaBCre/1072  "Wheel:Hub_Carrier_Vz:R2"
  adaDemux/1073 -> adaBCre/1073  "Wheel:hub_center_accx:front_left"
  adaDemux/1074 -> adaBCre/1074  "Wheel:hub_center_accx:front_right"
  adaDemux/1075 -> adaBCre/1075  "Wheel:hub_center_accx:rear_left"
  adaDemux/1076 -> adaBCre/1076  "Wheel:hub_center_accx:rear_right"
  adaDemux/1077 -> adaBCre/1077  "Wheel:hub_center_accy:front_left"
  adaDemux/1078 -> adaBCre/1078  "Wheel:hub_center_accy:front_right"
  adaDemux/1079 -> adaBCre/1079  "Wheel:hub_center_accy:rear_left"
  adaDemux/1080 -> adaBCre/1080  "Wheel:hub_center_accy:rear_right"
  adaDemux/1081 -> adaBCre/1081  "Wheel:hub_center_accz:front_left"
  adaDemux/1082 -> adaBCre/1082  "Wheel:hub_center_accz:front_right"
  adaDemux/1083 -> adaBCre/1083  "Wheel:hub_center_accz:rear_left"
  adaDemux/1084 -> adaBCre/1084  "Wheel:hub_center_accz:rear_right"
  adaDemux/1085 -> adaBCre/1085  "Wheel:Inclination:L1"
  adaDemux/1086 -> adaBCre/1086  "Wheel:Inclination:L2"
  adaDemux/1087 -> adaBCre/1087  "Wheel:Inclination:R1"
  adaDemux/1088 -> adaBCre/1088  "Wheel:Inclination:R2"
  adaDemux/1089 -> adaBCre/1089  "Wheel:Kingpin_Moment:L1"
  adaDemux/1090 -> adaBCre/1090  "Wheel:Kingpin_Moment:R1"
  adaDemux/1091 -> adaBCre/1091  "Wheel:Omega:L1"
  adaDemux/1092 -> adaBCre/1092  "Wheel:Omega:L2"
  adaDemux/1093 -> adaBCre/1093  "Wheel:Omega:R1"
  adaDemux/1094 -> adaBCre/1094  "Wheel:Omega:R2"
  adaDemux/1095 -> adaBCre/1095  "Wheel:Phi:L1"
  adaDemux/1096 -> adaBCre/1096  "Wheel:Phi:L2"
  adaDemux/1097 -> adaBCre/1097  "Wheel:Phi:R1"
  adaDemux/1098 -> adaBCre/1098  "Wheel:Phi:R2"
  adaDemux/1099 -> adaBCre/1099  "Wheel:Pitch:L1"
  adaDemux/1100 -> adaBCre/1100  "Wheel:Pitch:L2"
  adaDemux/1101 -> adaBCre/1101  "Wheel:Pitch:R1"
  adaDemux/1102 -> adaBCre/1102  "Wheel:Pitch:R2"
  adaDemux/1103 -> adaBCre/1103  "Wheel:Psi:L1"
  adaDemux/1104 -> adaBCre/1104  "Wheel:Psi:L2"
  adaDemux/1105 -> adaBCre/1105  "Wheel:Psi:R1"
  adaDemux/1106 -> adaBCre/1106  "Wheel:Psi:R2"
  adaDemux/1107 -> adaBCre/1107  "Wheel:Rotation:L1"
  adaDemux/1108 -> adaBCre/1108  "Wheel:Rotation:L2"
  adaDemux/1109 -> adaBCre/1109  "Wheel:Rotation:R1"
  adaDemux/1110 -> adaBCre/1110  "Wheel:Rotation:R2"
  adaDemux/1111 -> adaBCre/1111  "Wheel:Side_View_Angle:L1"
  adaDemux/1112 -> adaBCre/1112  "Wheel:Side_View_Angle:L2"
  adaDemux/1113 -> adaBCre/1113  "Wheel:Side_View_Angle:R1"
  adaDemux/1114 -> adaBCre/1114  "Wheel:Side_View_Angle:R2"
  adaDemux/1115 -> adaBCre/1115  "Wheel:Spindle_Steer:L1"
  adaDemux/1116 -> adaBCre/1116  "Wheel:Spindle_Steer:L2"
  adaDemux/1117 -> adaBCre/1117  "Wheel:Spindle_Steer:R1"
  adaDemux/1118 -> adaBCre/1118  "Wheel:Spindle_Steer:R2"
  adaDemux/1119 -> adaBCre/1119  "Wheel:Theta:L1"
  adaDemux/1120 -> adaBCre/1120  "Wheel:Theta:L2"
  adaDemux/1121 -> adaBCre/1121  "Wheel:Theta:R1"
  adaDemux/1122 -> adaBCre/1122  "Wheel:Theta:R2"
  adaDemux/1123 -> adaBCre/1123  "Wheel:wheel_center_dispx:front_left"
  adaDemux/1124 -> adaBCre/1124  "Wheel:wheel_center_dispx:front_right"
  adaDemux/1125 -> adaBCre/1125  "Wheel:wheel_center_dispx:rear_left"
  adaDemux/1126 -> adaBCre/1126  "Wheel:wheel_center_dispx:rear_right"
  adaDemux/1127 -> adaBCre/1127  "Wheel:wheel_center_dispy:front_left"
  adaDemux/1128 -> adaBCre/1128  "Wheel:wheel_center_dispy:front_right"
  adaDemux/1129 -> adaBCre/1129  "Wheel:wheel_center_dispy:rear_left"
  adaDemux/1130 -> adaBCre/1130  "Wheel:wheel_center_dispy:rear_right"
  adaDemux/1131 -> adaBCre/1131  "Wheel:wheel_center_dispz:front_left"
  adaDemux/1132 -> adaBCre/1132  "Wheel:wheel_center_dispz:front_right"
  adaDemux/1133 -> adaBCre/1133  "Wheel:wheel_center_dispz:rear_left"
  adaDemux/1134 -> adaBCre/1134  "Wheel:wheel_center_dispz:rear_right"
  adaDemux/1135 -> adaBCre/1135  "Wheel:Yaw:L1"
  adaDemux/1136 -> adaBCre/1136  "Wheel:Yaw:L2"
  adaDemux/1137 -> adaBCre/1137  "Wheel:Yaw:R1"
  adaDemux/1138 -> adaBCre/1138  "Wheel:Yaw:R2"
  adaDemux/1139 -> adaBCre/1139  "wheel_angles:camber_L1"
  adaDemux/1140 -> adaBCre/1140  "wheel_angles:camber_L2"
  adaDemux/1141 -> adaBCre/1141  "wheel_angles:camber_R1"
  adaDemux/1142 -> adaBCre/1142  "wheel_angles:camber_R2"
  adaDemux/1143 -> adaBCre/1143  "wheel_angles:camber_wrt_road_L1"
  adaDemux/1144 -> adaBCre/1144  "wheel_angles:camber_wrt_road_L2"
  adaDemux/1145 -> adaBCre/1145  "wheel_angles:camber_wrt_road_R1"
  adaDemux/1146 -> adaBCre/1146  "wheel_angles:camber_wrt_road_R2"
  adaDemux/1147 -> adaBCre/1147  "wheel_angles:caster_L1"
  adaDemux/1148 -> adaBCre/1148  "wheel_angles:caster_L2"
  adaDemux/1149 -> adaBCre/1149  "wheel_angles:caster_R1"
  adaDemux/1150 -> adaBCre/1150  "wheel_angles:caster_R2"
  adaDemux/1151 -> adaBCre/1151  "wheel_angles:caster_wrt_road_L1"
  adaDemux/1152 -> adaBCre/1152  "wheel_angles:caster_wrt_road_L2"
  adaDemux/1153 -> adaBCre/1153  "wheel_angles:caster_wrt_road_R1"
  adaDemux/1154 -> adaBCre/1154  "wheel_angles:caster_wrt_road_R2"
  adaDemux/1155 -> adaBCre/1155  "wheel_angles:toe_L1"
  adaDemux/1156 -> adaBCre/1156  "wheel_angles:toe_L2"
  adaDemux/1157 -> adaBCre/1157  "wheel_angles:toe_R1"
  adaDemux/1158 -> adaBCre/1158  "wheel_angles:toe_R2"
  adaDemux/1159 -> adaBCre/1159  "wheel_angles:toe_wrt_road_L1"
  adaDemux/1160 -> adaBCre/1160  "wheel_angles:toe_wrt_road_L2"
  adaDemux/1161 -> adaBCre/1161  "wheel_angles:toe_wrt_road_R1"
  adaDemux/1162 -> adaBCre/1162  "wheel_angles:toe_wrt_road_R2"
  adaDemux/1163 -> adaBCre/1163  "whl_front_wheel_XFORM:FX"
  adaDemux/1164 -> adaBCre/1164  "whl_front_wheel_XFORM:FY"
  adaDemux/1165 -> adaBCre/1165  "whl_front_wheel_XFORM:FZ"
  adaDemux/1166 -> adaBCre/1166  "whl_front_wheel_XFORM:Phi"
  adaDemux/1167 -> adaBCre/1167  "whl_front_wheel_XFORM:Psi"
  adaDemux/1168 -> adaBCre/1168  "whl_front_wheel_XFORM:Theta"
  adaDemux/1169 -> adaBCre/1169  "whl_front_wheel_XFORM:X"
  adaDemux/1170 -> adaBCre/1170  "whl_front_wheel_XFORM:Y"
  adaDemux/1171 -> adaBCre/1171  "whl_front_wheel_XFORM:Z"
  adaDemux/1172 -> adaBCre/1172  "whl_rear_wheel_XFORM:FX"
  adaDemux/1173 -> adaBCre/1173  "whl_rear_wheel_XFORM:FY"
  adaDemux/1174 -> adaBCre/1174  "whl_rear_wheel_XFORM:FZ"
  adaDemux/1175 -> adaBCre/1175  "whl_rear_wheel_XFORM:Phi"
  adaDemux/1176 -> adaBCre/1176  "whl_rear_wheel_XFORM:Psi"
  adaDemux/1177 -> adaBCre/1177  "whl_rear_wheel_XFORM:Theta"
  adaDemux/1178 -> adaBCre/1178  "whl_rear_wheel_XFORM:X"
  adaDemux/1179 -> adaBCre/1179  "whl_rear_wheel_XFORM:Y"
  adaDemux/1180 -> adaBCre/1180  "whl_rear_wheel_XFORM:Z"
  adaDemux/1181 -> adaBCre/1181  "whl_twin_rear_wheel_XFORM:FX"
  adaDemux/1182 -> adaBCre/1182  "whl_twin_rear_wheel_XFORM:FY"
  adaDemux/1183 -> adaBCre/1183  "whl_twin_rear_wheel_XFORM:FZ"
  adaDemux/1184 -> adaBCre/1184  "whl_twin_rear_wheel_XFORM:Phi"
  adaDemux/1185 -> adaBCre/1185  "whl_twin_rear_wheel_XFORM:Psi"
  adaDemux/1186 -> adaBCre/1186  "whl_twin_rear_wheel_XFORM:Theta"
  adaDemux/1187 -> adaBCre/1187  "whl_twin_rear_wheel_XFORM:X"
  adaDemux/1188 -> adaBCre/1188  "whl_twin_rear_wheel_XFORM:Y"
  adaDemux/1189 -> adaBCre/1189  "whl_twin_rear_wheel_XFORM:Z"
  adaDemux/1190 -> adaBCre/1190  "whr_front_wheel_XFORM:FX"
  adaDemux/1191 -> adaBCre/1191  "whr_front_wheel_XFORM:FY"
  adaDemux/1192 -> adaBCre/1192  "whr_front_wheel_XFORM:FZ"
  adaDemux/1193 -> adaBCre/1193  "whr_front_wheel_XFORM:Phi"
  adaDemux/1194 -> adaBCre/1194  "whr_front_wheel_XFORM:Psi"
  adaDemux/1195 -> adaBCre/1195  "whr_front_wheel_XFORM:Theta"
  adaDemux/1196 -> adaBCre/1196  "whr_front_wheel_XFORM:X"
  adaDemux/1197 -> adaBCre/1197  "whr_front_wheel_XFORM:Y"
  adaDemux/1198 -> adaBCre/1198  "whr_front_wheel_XFORM:Z"
  adaDemux/1199 -> adaBCre/1199  "whr_rear_wheel_XFORM:FX"
  adaDemux/1200 -> adaBCre/1200  "whr_rear_wheel_XFORM:FY"
  adaDemux/1201 -> adaBCre/1201  "whr_rear_wheel_XFORM:FZ"
  adaDemux/1202 -> adaBCre/1202  "whr_rear_wheel_XFORM:Phi"
  adaDemux/1203 -> adaBCre/1203  "whr_rear_wheel_XFORM:Psi"
  adaDemux/1204 -> adaBCre/1204  "whr_rear_wheel_XFORM:Theta"
  adaDemux/1205 -> adaBCre/1205  "whr_rear_wheel_XFORM:X"
  adaDemux/1206 -> adaBCre/1206  "whr_rear_wheel_XFORM:Y"
  adaDemux/1207 -> adaBCre/1207  "whr_rear_wheel_XFORM:Z"
  adaDemux/1208 -> adaBCre/1208  "whr_twin_rear_wheel_XFORM:FX"
  adaDemux/1209 -> adaBCre/1209  "whr_twin_rear_wheel_XFORM:FY"
  adaDemux/1210 -> adaBCre/1210  "whr_twin_rear_wheel_XFORM:FZ"
  adaDemux/1211 -> adaBCre/1211  "whr_twin_rear_wheel_XFORM:Phi"
  adaDemux/1212 -> adaBCre/1212  "whr_twin_rear_wheel_XFORM:Psi"
  adaDemux/1213 -> adaBCre/1213  "whr_twin_rear_wheel_XFORM:Theta"
  adaDemux/1214 -> adaBCre/1214  "whr_twin_rear_wheel_XFORM:X"
  adaDemux/1215 -> adaBCre/1215  "whr_twin_rear_wheel_XFORM:Y"
  adaDemux/1216 -> adaBCre/1216  "whr_twin_rear_wheel_XFORM:Z"
  adaDemux/1217 -> adaBCre/1217  "Steering_Column:steering_assist_force"
  adaDemux/1218 -> adaBCre/1218  "Steering_Column:steering_assist_torque"
  adaDemux/1219 -> adaBCre/1219  "Steering_Column:lower_column_rotation"
  adaDemux/1220 -> adaBCre/1220  "Steering_Column:lower_column_rotational_velocity"
  adaDemux/1221 -> adaBCre/1221  "Steering_Column:friction_torque"
  adaDemux/1222 -> adaBCre/1222  "Steering_Column:upper_cardan_shaft_ratio"
  adaDemux/1223 -> adaBCre/1223  "Steering_Column:middle_cardan_shaft_ratio"
  adaDemux/1224 -> adaBCre/1224  "Steering_Column:lower_cardan_shaft_ratio"
  adaDemux/1225 -> adaBCre/1225  "Steering_Column:overall_cardan_shaft_ratio"
  adaDemux/1226 -> adaBCre/1226  "Steering_Column:inertial_torque"
  adaDemux/1227 -> adaBCre/1227  "Steering_Column:steering_wheel_torque"
  adaDemux/1228 -> adaBCre/1228  "Steering_Column:steering_wheel_torque_without_upper_inertia"
  adaDemux/1229 -> adaBCre/1229  "Steering_Column:lower_column_deformation"
  adaDemux/1230 -> adaBCre/1230  "Steering_Column:lower_column_deformation_velocity"
  adaDemux/1231 -> adaBCre/1231  "Steering_Column:upper_column_deformation"
  adaDemux/1232 -> adaBCre/1232  "Steering_Column:upper_column_deformation_velocity"
  adaDemux/1233 -> adaBCre/1233  "Steering_Column:lower_column_stiffness_torque"
  adaDemux/1234 -> adaBCre/1234  "Steering_Column:lower_column_damping_torque"
  adaDemux/1235 -> adaBCre/1235  "Steering_Column:upper_column_stiffness_torque"
  adaDemux/1236 -> adaBCre/1236  "Steering_Column:upper_column_damping_torque"
  adaDemux/1237 -> adaBCre/1237  "Steering_Column:total_torque_upper_column"
  adaDemux/1238 -> adaBCre/1238  "Steering_Column:total_torque_lower_column"
  adaDemux/1239 -> adaBCre/1239  "Steering_Column:hardy_disc_deformation"
  adaDemux/1240 -> adaBCre/1240  "Steering_Column:upper_column_angle"
  adaDemux/1241 -> adaBCre/1241  "Steering_Column:upper_column_velocity"
  adaDemux/1242 -> adaBCre/1242  "Steering_Column:lower_cardan_joint_output_rotation"
  adaDemux/1243 -> adaBCre/1243  "Steering_Column:lower_cardan_joint_output_velocity"
  adaDemux/1244 -> adaBCre/1244  "Steering_Column:middle_cardan_joint_output_rotation"
  adaDemux/1245 -> adaBCre/1245  "Steering_Column:middle_cardan_joint_output_velocity"
  adaDemux/1246 -> adaBCre/1246  "Steering_Column:upper_cardan_joint_output_rotation"
  adaDemux/1247 -> adaBCre/1247  "Steering_Column:upper_cardan_joint_output_velocity"
  adaDemux/1248 -> adaBCre/1248  "Steering_Column:simulator_steering_wheel_torque"
  adaDemux/1249 -> adaBCre/1249  "Steering_Torsion_Bar:torsion_bar_twist_angle"
  adaDemux/1250 -> adaBCre/1250  "Steering_Torsion_Bar:friction_torque"
  adaDemux/1251 -> adaBCre/1251  "Steering_Torsion_Bar:torsion_bar_twist_angle_saturated"
  adaDemux/1252 -> adaBCre/1252  "Steering_Torsion_Bar:torsion_bar_deformation_velocity"
  adaDemux/1253 -> adaBCre/1253  "Steering_Torsion_Bar:torsion_bar_load"
  adaDemux/1254 -> adaBCre/1254  "Steering_Rack_Pinion:rack_displacement_saturated"
  adaDemux/1255 -> adaBCre/1255  "Steering_Rack_Pinion:pinion_rotation"
  adaDemux/1256 -> adaBCre/1256  "Steering_Rack_Pinion:pinion_rotational_velocity"
  adaDemux/1257 -> adaBCre/1257  "Steering_Rack_Pinion:rack_force_from_lower_column"
  adaDemux/1258 -> adaBCre/1258  "Steering_Rack_Pinion:rack_friction_force"
  adaDemux/1259 -> adaBCre/1259  "Steering_Rack_Pinion:rack_acceleration"
  adaDemux/1260 -> adaBCre/1260  "Steering_Rack_Pinion:total_rack_mass"
  adaDemux/1261 -> adaBCre/1261  "Steering_Rack_Pinion:rack_total_force"
  adaDemux/1262 -> adaBCre/1262  "Steering_Rack_Pinion:rack_velocity"
  adaDemux/1263 -> adaBCre/1263  "Steering_Rack_Pinion:rack_force"
  adaDemux/1264 -> adaBCre/1264  "Steering_Rack_Pinion:rack_displacement"
  adaDemux/1265 -> adaBCre/1265  "Motor:motor_angle"
  adaDemux/1266 -> adaBCre/1266  "Motor:motor_velocity"
  adaDemux/1267 -> adaBCre/1267  "Motor:motor_torque"
  adaDemux/1268 -> adaBCre/1268  "Motor:motor_current"
  adaDemux/1269 -> adaBCre/1269  "Motor:motor_friction"
  adaDemux/1270 -> adaBCre/1270  "path_sensor:total_lap_time"
  adaDemux/1271 -> adaBCre/1271  "path_sensor:total_lap_count"
  adaDemux/1272 -> adaBCre/1272  "path_sensor:last_sector_time"
  adaDemux/1273 -> adaBCre/1273  "path_sensor:progressive_time"
  adaDemux/1274 -> adaBCre/1274  "path_sensor:path_s"
  adaDemux/1275 -> adaBCre/1275  "path_sensor:path_distance"
  adaDemux/1276 -> adaBCre/1276  "Animator_Widget:longitudinal_speed"
  adaDemux/1277 -> adaBCre/1277  "Animator_Widget:engine_rpm"
  adaDemux/1278 -> adaBCre/1278  "ges_hub_XFORMFL:X"
  adaDemux/1279 -> adaBCre/1279  "ges_hub_XFORMFL:Y"
  adaDemux/1280 -> adaBCre/1280  "ges_hub_XFORMFL:Z"
  adaDemux/1281 -> adaBCre/1281  "ges_hub_XFORMFL:Psi"
  adaDemux/1282 -> adaBCre/1282  "ges_hub_XFORMFL:Theta"
  adaDemux/1283 -> adaBCre/1283  "ges_hub_XFORMFL:Phi"
  adaDemux/1284 -> adaBCre/1284  "hub2cp_XFORMFL:X"
  adaDemux/1285 -> adaBCre/1285  "hub2cp_XFORMFL:Y"
  adaDemux/1286 -> adaBCre/1286  "hub2cp_XFORMFL:Z"
  adaDemux/1287 -> adaBCre/1287  "cp_force_longitudinalFL:X"
  adaDemux/1288 -> adaBCre/1288  "cp_force_longitudinalFL:Y"
  adaDemux/1289 -> adaBCre/1289  "cp_force_longitudinalFL:Z"
  adaDemux/1290 -> adaBCre/1290  "cp_force_lateralFL:X"
  adaDemux/1291 -> adaBCre/1291  "cp_force_lateralFL:Y"
  adaDemux/1292 -> adaBCre/1292  "cp_force_lateralFL:Z"
  adaDemux/1293 -> adaBCre/1293  "cp_force_normalFL:X"
  adaDemux/1294 -> adaBCre/1294  "cp_force_normalFL:Y"
  adaDemux/1295 -> adaBCre/1295  "cp_force_normalFL:Z"
  adaDemux/1296 -> adaBCre/1296  "ges_hub_XFORMFR:X"
  adaDemux/1297 -> adaBCre/1297  "ges_hub_XFORMFR:Y"
  adaDemux/1298 -> adaBCre/1298  "ges_hub_XFORMFR:Z"
  adaDemux/1299 -> adaBCre/1299  "ges_hub_XFORMFR:Psi"
  adaDemux/1300 -> adaBCre/1300  "ges_hub_XFORMFR:Theta"
  adaDemux/1301 -> adaBCre/1301  "ges_hub_XFORMFR:Phi"
  adaDemux/1302 -> adaBCre/1302  "hub2cp_XFORMFR:X"
  adaDemux/1303 -> adaBCre/1303  "hub2cp_XFORMFR:Y"
  adaDemux/1304 -> adaBCre/1304  "hub2cp_XFORMFR:Z"
  adaDemux/1305 -> adaBCre/1305  "cp_force_longitudinalFR:X"
  adaDemux/1306 -> adaBCre/1306  "cp_force_longitudinalFR:Y"
  adaDemux/1307 -> adaBCre/1307  "cp_force_longitudinalFR:Z"
  adaDemux/1308 -> adaBCre/1308  "cp_force_lateralFR:X"
  adaDemux/1309 -> adaBCre/1309  "cp_force_lateralFR:Y"
  adaDemux/1310 -> adaBCre/1310  "cp_force_lateralFR:Z"
  adaDemux/1311 -> adaBCre/1311  "cp_force_normalFR:X"
  adaDemux/1312 -> adaBCre/1312  "cp_force_normalFR:Y"
  adaDemux/1313 -> adaBCre/1313  "cp_force_normalFR:Z"
  adaDemux/1314 -> adaBCre/1314  "ges_hub_XFORMRL:X"
  adaDemux/1315 -> adaBCre/1315  "ges_hub_XFORMRL:Y"
  adaDemux/1316 -> adaBCre/1316  "ges_hub_XFORMRL:Z"
  adaDemux/1317 -> adaBCre/1317  "ges_hub_XFORMRL:Psi"
  adaDemux/1318 -> adaBCre/1318  "ges_hub_XFORMRL:Theta"
  adaDemux/1319 -> adaBCre/1319  "ges_hub_XFORMRL:Phi"
  adaDemux/1320 -> adaBCre/1320  "hub2cp_XFORMRL:X"
  adaDemux/1321 -> adaBCre/1321  "hub2cp_XFORMRL:Y"
  adaDemux/1322 -> adaBCre/1322  "hub2cp_XFORMRL:Z"
  adaDemux/1323 -> adaBCre/1323  "cp_force_longitudinalRL:X"
  adaDemux/1324 -> adaBCre/1324  "cp_force_longitudinalRL:Y"
  adaDemux/1325 -> adaBCre/1325  "cp_force_longitudinalRL:Z"
  adaDemux/1326 -> adaBCre/1326  "cp_force_lateralRL:X"
  adaDemux/1327 -> adaBCre/1327  "cp_force_lateralRL:Y"
  adaDemux/1328 -> adaBCre/1328  "cp_force_lateralRL:Z"
  adaDemux/1329 -> adaBCre/1329  "cp_force_normalRL:X"
  adaDemux/1330 -> adaBCre/1330  "cp_force_normalRL:Y"
  adaDemux/1331 -> adaBCre/1331  "cp_force_normalRL:Z"
  adaDemux/1332 -> adaBCre/1332  "ges_hub_XFORMRR:X"
  adaDemux/1333 -> adaBCre/1333  "ges_hub_XFORMRR:Y"
  adaDemux/1334 -> adaBCre/1334  "ges_hub_XFORMRR:Z"
  adaDemux/1335 -> adaBCre/1335  "ges_hub_XFORMRR:Psi"
  adaDemux/1336 -> adaBCre/1336  "ges_hub_XFORMRR:Theta"
  adaDemux/1337 -> adaBCre/1337  "ges_hub_XFORMRR:Phi"
  adaDemux/1338 -> adaBCre/1338  "hub2cp_XFORMRR:X"
  adaDemux/1339 -> adaBCre/1339  "hub2cp_XFORMRR:Y"
  adaDemux/1340 -> adaBCre/1340  "hub2cp_XFORMRR:Z"
  adaDemux/1341 -> adaBCre/1341  "cp_force_longitudinalRR:X"
  adaDemux/1342 -> adaBCre/1342  "cp_force_longitudinalRR:Y"
  adaDemux/1343 -> adaBCre/1343  "cp_force_longitudinalRR:Z"
  adaDemux/1344 -> adaBCre/1344  "cp_force_lateralRR:X"
  adaDemux/1345 -> adaBCre/1345  "cp_force_lateralRR:Y"
  adaDemux/1346 -> adaBCre/1346  "cp_force_lateralRR:Z"
  adaDemux/1347 -> adaBCre/1347  "cp_force_normalRR:X"
  adaDemux/1348 -> adaBCre/1348  "cp_force_normalRR:Y"
  adaDemux/1349 -> adaBCre/1349  "cp_force_normalRR:Z"
  adaDemux/1350 -> adaBCre/1350  "Road_Material:front_left_tire"
  adaDemux/1351 -> adaBCre/1351  "Road_Material:front_right_tire"
  adaDemux/1352 -> adaBCre/1352  "Road_Material:rear_left_tire"
  adaDemux/1353 -> adaBCre/1353  "Road_Material:rear_right_tire"
  adaBCre/1 -> outputBus/1
